simulink model "ndtm_V2"  (R2018b)
settings: configuration reference "Physics" (kept outside this file)
model workspace (MAT data in the model file):
  x0_initialstates = [0 0 0 0 0 0]
undefined symbols (not defined in the file): F0z, h, INIT__initialvalues__Vehicle_InitialPitchRate_radps, INIT__initialvalues__Vehicle_InitialRollRate_radps, INIT__initialvalues__Vehicle_InitialVelocity_mps__1, INIT__initialvalues__Vehicle_InitialVelocity_mps__2, INIT__initialvalues__Vehicle_InitialVelocity_mps__3, INIT__initialvalues__Vehicle_InitialYawRate_radps, SUS__Antisway__c_AntiSwayTSpringFrRe_Nmprad__1, SUS__Antisway__c_AntiSwayTSpringFrRe_Nmprad__2, SUS__Antisway__phi_AntiSwayNeutralAngleFrRe_rad__1, SUS__Antisway__phi_AntiSwayNeutralAngleFrRe_rad__2, SUS__Antisway__r_AntiSwayArmRadiusFrRe_m__1, SUS__Antisway__r_AntiSwayArmRadiusFrRe_m__2, SUS__Compliance__Cz_DamperRateFrRe_Nspm__1, SUS__Compliance__Cz_DamperRateFrRe_Nspm__2, SUS__Compliance__cz_SpringRateFrRe_Npm__1, SUS__Compliance__cz_SpringRateFrRe_Npm__2, SUS__Compliance__F0z_SpringPreloadFrRe_N__1, SUS__Compliance__F0z_SpringPreloadFrRe_N__2, SUS__Compliance__h_InertialFrameOffset_COGtoAxle_m, SUS__Kinematics__k_CamberATSteerCenterF__1, SUS__Kinematics__k_CamberATSteerCenterF__2, SUS__Kinematics__k_CamberVSHeightFrRe__1, SUS__Kinematics__k_CamberVSHeightFrRe__2, SUS__Kinematics__k_CasterATSteerCenterF__1, SUS__Kinematics__k_CasterATSteerCenterF__2, SUS__Kinematics__k_CasterVSHeightFrRe__1, SUS__Kinematics__k_CasterVSHeightFrRe__2, SUS__Kinematics__k_RollSteerVSHeightFrRe_radpm__1, SUS__Kinematics__k_RollSteerVSHeightFrRe_radpm__2, SUS__Kinematics__nu0_ToeATSteerCenterFrRe_rad__1, SUS__Kinematics__nu0_ToeATSteerCenterFrRe_rad__2, tireFL__SCALING__LFZO, tireFR__SCALING__LFZO, tireRL__SCALING__LFZO, tireRR__SCALING__LFZO, VEH, VEH__Aerodynamics__beta_wind_end_rad, VEH__Aerodynamics__beta_wind_start_rad, VEH__Aerodynamics__beta_wind_step_rad, VEH__Aerodynamics__cl_LongitudinalLift, VEH__Aerodynamics__Cs_LatDragCoeff_end, VEH__Aerodynamics__Cs_LatDragCoeff_start, VEH__Aerodynamics__Cs_LatDragCoeff_step, VEH__Aerodynamics__Cym_DragYawMomentCoeff_end, VEH__Aerodynamics__Cym_DragYawMomentCoeff_start, VEH__Aerodynamics__Cym_DragYawMomentCoeff_step, VEH__Environment__a_Gravity_mps2, VEH__Tires__p_Tires_pa__1, VEH__Tires__p_Tires_pa__2, VEH__Tires__p_Tires_pa__3, VEH__Tires__p_Tires_pa__4, VEH__VehicleData__l_WheelbaseF_m, VEH__VehicleData__l_WheelbaseTotal_m, VEH__VehicleData__m_Vehicle_kg, VEH__VehicleData__w_GeomCenterlineToCOG_m, VEH__VehicleData__w_TrackF_m, VEH__VehicleData__w_TrackR_m
libraries: vehdynlibsuspension x7, vehdynlibtire x4, vehdynlibtire_TUM x4, autolibutils x2, sharedtransform x2, vehdynlibeom_TUM x1
(part 3 of 4)

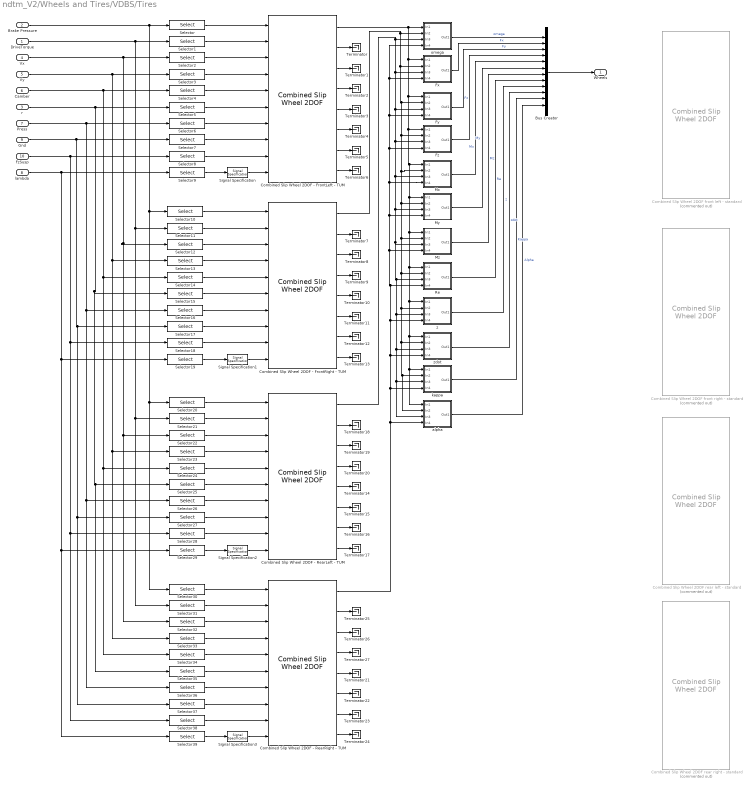
== system ndtm_V2/Wheels and Tires/VDBS/Tires ==
  DriveTorque : Inport
  Brake Pressure : Inport  Port=2
  r : Inport  Port=3
  Vx : Inport  Port=4
  Vy : Inport  Port=5
  Camber : Inport  Port=6
  Press : Inport  Port=7  Unit=Pa
  lambda : Inport  Port=8  Unit=1
  Gnd : Inport  Port=9
  FzSusp : Inport  Port=10
  Bus Creator : BusCreator  Inputs=12
  Combined Slip Wheel 2DOF front left - standard : vehdynlibtire/Combined Slip Wheel 2DOF  Commented=on  BrakeType=Disc  mu_static=0.6  mu_kinetic=0.6  disk_abore=.08  Rm=0.1475  num_pads=1  drum_abore=0.0508  drum_a=0.123  drum_c=0.212  drum_r=0.15  drum_theta1=0  drum_theta2=126  brake_p_bpt=[1 11.4736842105263 21.9473684210526 32.4210526315789 42.8947368421053 53.3684210526316 63.8421052631579 74.3157894736842 84.7894736842105 95.2631578947368 105.736842105263 116.210526315789 126.684210526316 137.157894736842 147.631578947368 158.105263157895 168.578947368421 179.052631578947 189.526315789474 200]  brake_n_bpt=[0 52.6315789473684 105.263157894737 157.894736842105 210.526315789474 263.157894736842 315.789473684211 368.421052631579 421.052631578947 473.684210526316 526.315789473684 578.947368421053 631.578947368421 684.210526315789 736.842105263158 789.473684210526 842.105263157895 894.736842105263 947.368421052632 1000]  f_brake_t=[43.4900602404453 42.5056030554862 41.5350898940194 40.5780454442085 39.6340111501808 38.7025443887544 37.7832176914519 36.8756180088306 35.9793460143796 35.0940154454303 34.2192524787115 33.3546951383474 32.4999927342521 31.6548053290159 30.8188032315107 29.991666515561 29.1730845621415 28.362755623661 27.5603864089927 26.765691687993;498.991217495636 487.695866636631 476.560505099801 465.579679307235 454.748127933653 444.060772460445 433.51270824929 423.099196101319 412.81565427025 402.657650900201 392.620896861006 382.701238955775 372.894653477208 363.197240090814 353.605216024701 344.114910546964 334.722759712992 325.425301366216 316.219170376863 307.10109410434;954.492374750826 932.886130217776 911.585920305583 890.581313170261 869.862244717126 849.419000532136 829.242198807128 809.322774193808 789.651962526121 770.221286354971 751.0225412433 732.047782773203 713.289314220164 694.739674852612 676.391628817892 658.238154578366 640.272434863842 622.48784710877 604.877954344734 587.436496520688;1409.99353200602 1378.07639379892 1346.61133551136 1315.58294703329 1284.9763615006 1254.77722860383 1224.97168936497 1195.5463522863 1166.48827078199 1137.78492180974 1109.42418562559 1081.39432659063 1053.68397496312 1026.28210961441 999.178041611083 972.361398609768 945.822110014692 919.550392851325 893.536738312604 867.771898937035;1865.49468926121 1823.26665738007 1781.63675071715 1740.58458089631 1700.09047828407 1660.13545667552 1620.7011799228 1581.76993037878 1543.32457903786 1505.34855726451 1467.82583000789 1430.74087040806 1394.07863570608 1357.82454437621 1321.96445440427 1286.48464264117 1251.37178516554 1216.61293859388 1182.19552228048 1148.10730135338;2320.9958465164 2268.45692096121 2216.66216592293 2165.58621475934 2115.20459506754 2065.49368474721 2016.43067048064 1967.99350847127 1920.16088729373 1872.91219271928 1826.22747439018 1780.08741422549 1734.47329644903 1689.36697913801 1644.75086719747 1600.60788667257 1556.92146031639 1513.67548433643 1470.85430624835 1428.44270376973;2776.49700377159 2713.64718454235 2651.68758112871 2590.58784862237 2530.31871185102 2470.8519128189 2412.16016103848 2354.21708656376 2296.9971955496 2240.47582817405 2184.62911877248 2129.43395804292 2074.86795719199 2020.9094138998 1967.53727999066 1914.73113070398 1862.47113546724 1810.73803007899 1759.51309021622 1708.77810618608;3231.99816102678 3158.8374481235 3086.71299633449 3015.58948248539 2945.43282863449 2876.21014089059 2807.88965159632 2740.44066465625 2673.83350380547 2608.03946362882 2543.03076315477 2478.78050186034 2415.26261793494 2352.4518486616 2290.32369278385 2228.85437473538 2168.02081061809 2107.80057582154 2048.17187418409 1989.11350860242;3687.49931828197 3604.02771170464 3521.73841154027 3440.59111634842 3360.54694541796 3281.56836896228 3203.61914215416 3126.66424274874 3050.66981206134 2975.60309908359 2901.43240753707 2828.12704567777 2755.6572786779 2683.9942834234 2613.11010557704 2542.97761876678 2473.57048576894 2404.8631215641 2336.83065815196 2269.44891101877;4143.00047553716 4049.21797528579 3956.76382674606 3865.59275021144 3775.66106220143 3686.92659703397 3599.34863271199 3512.88782084123 3427.50612031721 3343.16673453836 3259.83405191936 3177.4735894952 3096.05193942085 3015.5367181852 2935.89651837023 2857.10086279818 2779.12016091979 2701.92566730665 2625.48944211983 2549.78431343512;4598.50163279235 4494.40823886693 4391.78924195184 4290.59438407447 4190.77517898491 4092.28482510566 3995.07812326983 3899.11139893372 3804.34242857308 3710.73036999313 3618.23569630166 3526.82013331263 3436.44660016381 3347.079152947 3258.68293116342 3171.22410682959 3084.66983607064 2998.98821304921 2914.1482260877 2830.11971585147;5054.00279004754 4939.59850244808 4826.81465715762 4715.59601793749 4605.88929576838 4497.64305317735 4390.80761382767 4285.3349770262 4181.17873682896 4078.2940054479 3976.63734068395 3876.16667713006 3776.84126090677 3678.62158770879 3581.46934395661 3485.34735086099 ...(+2764 chars)]  tireParamSet=vdynPassCar.mat  plySteer=off  turnslip=off  PRESMAX=1000000  PRESMIN=10000  FZMAX=10000  FZMIN=100  VXLOW=0.1  KPUMAX=1.5  KPUMIN=-1.5  ALPMAX=1.5  ALPMIN=-1.5  CAMMAX=0.2  CAMMIN=-0.2  LONGVL=16.7  omegao=0  br=1e-3  UNLOADED_RADIUS=0.42  NOMPRES=224000  FNOMIN=4000  WIDTH=0.209  MASS=9.46+20  IYY=0.740633832792491  GRAVITY=-9.81  zo=.015  zdoto=0  BREFF=8.25094594147963  DREFF=0.260468730454265  FREFF=0.0735298544471851  Q_RE0=1.00866439868088  Q_V1=0.000760413786224011  Q_V2=0.0463384792019201  Q_FZ1=0  Q_FZ2=15.6870832810226  Q_FZ3=0  Q_FCX=0.138643970247602  Q_FCY=0.10843499565426  Q_FCY2=-0.465763352339538  PFZ1=0.69958166705601  VERTICAL_STIFFNESS=207885.061134007  VERTICAL_DAMPING=494.649255786991  LONGITUDINAL_STIFFNESS=388714.175879854  LATERAL_STIFFNESS=157087.404633332  PCFX1=0.18539229191199  PCFX2=0  PCFX3=0  PCFY1=0.163183345037677  PCFY2=0  PCFY3=0.249094918231954  Q_RA1=0.675942571700787  Q_RA2=0.73800463546164  Q_RB1=1.04487486456705  Q_RB2=-1.191763806629  PCX1=1.58523057950359  PDX1=1.0239116238178  PDX2=-0.0842405110022724  PDX3=0  PEX1=0.110312777158455  PEX2=0.313468516038146  PEX3=0  PEX4=0.0016060905760045  PKX1=21.3872544684023  PKX2=14.0006541873175  PKX3=-0.405326109653452  PHX1=0.000212599305364818  PHX2=0.00115950515263055  PVX1=1.59236164471432e-05  PVX2=0.000104321112127671  PPX1=-0.349461321276586  PPX2=0.387840040616429  PPX3=-0.0969947336569324  PPX4=0.0632271859795801  RBX1=12.7633329850276  RBX2=9.5787123658471  RBX3=0  RCX1=1.02796280922059  REX1=-0.45202516851367  REX2=-0.47304886171176  RHX1=0.000233272373115809  QSX1=-0.00788307788961443  QSX2=0.954629515459396  QSX3=0.0155855777667025  QSX4=0.125904607142414  QSX5=1.01110069703963  QSX6=20.1938577118433  QSX7=0.310818120717083  QSX8=-0.0430823751139655  QSX9=0.636494404888216  QSX10=0.142438060591663  QSX11=0.346766530036373  QSX12=0  QSX13=0  QSX14=0  PPMX1=0  PCY1=1.34299950037631  PDY1=0.878267729082195  PDY2=-0.0644597923147385  PDY3=0  PEY1=-0.809776534470972  PEY2=-0.600180598867198  PEY3=0.0991732552633487  PEY4=-6.5577974035573  PEY5=0  PKY1=-15.57  PKY2=1.73126522291751  PKY3=0.365349873517229  PKY4=1.98176755955416  PKY5=0  PKY6=-0.884005199550313  PKY7=-0.237259727611847  PHY1=-0.00183370557235628  PHY2=0.00346401302716671  PVY1=-0.00675427560163264  PVY2=0.036379218103843  PVY3=-0.163543984089166  PVY4=-0.491003349625726  PPY1=-0.62059646553185  PPY2=-0.0647824842338686  PPY3=-0.164648843290686  PPY4=0.283193909060098  PPY5=0  RBY1=10.7588809173639  RBY2=7.70420065295029  RBY3=3.40283755070691e-06  RBY4=0  RCY1=1.06691874059059  REY1=0.308244924574305  REY2=7.48775032604508e-06  RHY1=0.0118479204960415  RHY2=7.63650177161071e-06  RVY1=0.0560024425050078  RVY2=7.48487127056197e-06  RVY3=0  RVY4=98.4047026517149  RVY5=2.02759273900054  RVY6=15.7623064923347  QSY1=0.00699077564863536  QSY2=0  QSY3=0.00153535478298811  QSY4=8.55710322455322e-05  QSY5=0  QSY6=0  QSY7=0.89443879773793  QSY8=-0.403227641260894  QBZ1=11.666656027484  QBZ2=-1.30355438574485  QBZ3=0  QBZ4=0.177918305399071  QBZ5=-0.162481135068033  QBZ6=0  QBZ9=30.1445534682089  QBZ10=0  QCZ1=1.29026978207574  QDZ1=0.0886972644991399  QDZ2=-0.0058634820161856  QDZ3=0.3805597481383  QDZ4=0  QDZ6=0.00160914918118959  QDZ7=-0.00211036330862154  QDZ8=-0.13921904912557  QDZ9=0.00816585550028243  QDZ10=0  QDZ11=0  QEZ1=-2.19802254534746  QEZ2=1.01850535789165  QEZ3=0  QEZ4=0.278379679112054  QEZ5=-0.548414722765386  QHZ1=0.00148361198869669  QHZ2=0.00202017567585904  QHZ3=0.240316641332066  QHZ4=-0.210114035738085  PPZ1=-0.443927982388615  PPZ2=0  SSZ1=0.00914999585397887  SSZ2=0.0389830656052735  SSZ3=0  SSZ4=0  PDXP1=0.396718274678791  PDXP2=0  PDXP3=0  PKYP1=1.00587060633573  PDYP1=0.40483048923438  PDYP2=0  PDYP3=0  PDYP4=0  PHYP1=0.992731942067188  PHYP2=0.150352945499914  PHYP3=0  PHYP4=-3.98988682633674  PECP1=0.502379254513503  PECP2=0  QDTP1=10.0178654287947  QCRP1=0.200627747200702  QCRP2=0.0995735881599772  QBRP1=0.0997107127960717  QDRP1=1.01432910167423  QDRP2=0  aMode=2
      settings: SourceProductName=Vehicle Dynamics Blockset
  Combined Slip Wheel 2DOF front right - standard : vehdynlibtire/Combined Slip Wheel 2DOF  Commented=on  BrakeType=Disc  mu_static=0.6  mu_kinetic=0.6  disk_abore=0.08  Rm=0.1475  num_pads=1  drum_abore=0.0508  drum_a=0.123  drum_c=0.212  drum_r=0.15  drum_theta1=0  drum_theta2=126  brake_p_bpt=[1 11.4736842105263 21.9473684210526 32.4210526315789 42.8947368421053 53.3684210526316 63.8421052631579 74.3157894736842 84.7894736842105 95.2631578947368 105.736842105263 116.210526315789 126.684210526316 137.157894736842 147.631578947368 158.105263157895 168.578947368421 179.052631578947 189.526315789474 200]  brake_n_bpt=[0 52.6315789473684 105.263157894737 157.894736842105 210.526315789474 263.157894736842 315.789473684211 368.421052631579 421.052631578947 473.684210526316 526.315789473684 578.947368421053 631.578947368421 684.210526315789 736.842105263158 789.473684210526 842.105263157895 894.736842105263 947.368421052632 1000]  f_brake_t=[43.4900602404453 42.5056030554862 41.5350898940194 40.5780454442085 39.6340111501808 38.7025443887544 37.7832176914519 36.8756180088306 35.9793460143796 35.0940154454303 34.2192524787115 33.3546951383474 32.4999927342521 31.6548053290159 30.8188032315107 29.991666515561 29.1730845621415 28.362755623661 27.5603864089927 26.765691687993;498.991217495636 487.695866636631 476.560505099801 465.579679307235 454.748127933653 444.060772460445 433.51270824929 423.099196101319 412.81565427025 402.657650900201 392.620896861006 382.701238955775 372.894653477208 363.197240090814 353.605216024701 344.114910546964 334.722759712992 325.425301366216 316.219170376863 307.10109410434;954.492374750826 932.886130217776 911.585920305583 890.581313170261 869.862244717126 849.419000532136 829.242198807128 809.322774193808 789.651962526121 770.221286354971 751.0225412433 732.047782773203 713.289314220164 694.739674852612 676.391628817892 658.238154578366 640.272434863842 622.48784710877 604.877954344734 587.436496520688;1409.99353200602 1378.07639379892 1346.61133551136 1315.58294703329 1284.9763615006 1254.77722860383 1224.97168936497 1195.5463522863 1166.48827078199 1137.78492180974 1109.42418562559 1081.39432659063 1053.68397496312 1026.28210961441 999.178041611083 972.361398609768 945.822110014692 919.550392851325 893.536738312604 867.771898937035;1865.49468926121 1823.26665738007 1781.63675071715 1740.58458089631 1700.09047828407 1660.13545667552 1620.7011799228 1581.76993037878 1543.32457903786 1505.34855726451 1467.82583000789 1430.74087040806 1394.07863570608 1357.82454437621 1321.96445440427 1286.48464264117 1251.37178516554 1216.61293859388 1182.19552228048 1148.10730135338;2320.9958465164 2268.45692096121 2216.66216592293 2165.58621475934 2115.20459506754 2065.49368474721 2016.43067048064 1967.99350847127 1920.16088729373 1872.91219271928 1826.22747439018 1780.08741422549 1734.47329644903 1689.36697913801 1644.75086719747 1600.60788667257 1556.92146031639 1513.67548433643 1470.85430624835 1428.44270376973;2776.49700377159 2713.64718454235 2651.68758112871 2590.58784862237 2530.31871185102 2470.8519128189 2412.16016103848 2354.21708656376 2296.9971955496 2240.47582817405 2184.62911877248 2129.43395804292 2074.86795719199 2020.9094138998 1967.53727999066 1914.73113070398 1862.47113546724 1810.73803007899 1759.51309021622 1708.77810618608;3231.99816102678 3158.8374481235 3086.71299633449 3015.58948248539 2945.43282863449 2876.21014089059 2807.88965159632 2740.44066465625 2673.83350380547 2608.03946362882 2543.03076315477 2478.78050186034 2415.26261793494 2352.4518486616 2290.32369278385 2228.85437473538 2168.02081061809 2107.80057582154 2048.17187418409 1989.11350860242;3687.49931828197 3604.02771170464 3521.73841154027 3440.59111634842 3360.54694541796 3281.56836896228 3203.61914215416 3126.66424274874 3050.66981206134 2975.60309908359 2901.43240753707 2828.12704567777 2755.6572786779 2683.9942834234 2613.11010557704 2542.97761876678 2473.57048576894 2404.8631215641 2336.83065815196 2269.44891101877;4143.00047553716 4049.21797528579 3956.76382674606 3865.59275021144 3775.66106220143 3686.92659703397 3599.34863271199 3512.88782084123 3427.50612031721 3343.16673453836 3259.83405191936 3177.4735894952 3096.05193942085 3015.5367181852 2935.89651837023 2857.10086279818 2779.12016091979 2701.92566730665 2625.48944211983 2549.78431343512;4598.50163279235 4494.40823886693 4391.78924195184 4290.59438407447 4190.77517898491 4092.28482510566 3995.07812326983 3899.11139893372 3804.34242857308 3710.73036999313 3618.23569630166 3526.82013331263 3436.44660016381 3347.079152947 3258.68293116342 3171.22410682959 3084.66983607064 2998.98821304921 2914.1482260877 2830.11971585147;5054.00279004754 4939.59850244808 4826.81465715762 4715.59601793749 4605.88929576838 4497.64305317735 4390.80761382767 4285.3349770262 4181.17873682896 4078.2940054479 3976.63734068395 3876.16667713006 3776.84126090677 3678.62158770879 3581.46934395661 3485.34735086099 ...(+2764 chars)]  tireParamSet=vdynPassCar.mat  plySteer=off  turnslip=off  PRESMAX=1000000  PRESMIN=10000  FZMAX=10000  FZMIN=100  VXLOW=0.1  KPUMAX=1.5  KPUMIN=-1.5  ALPMAX=1.5  ALPMIN=-1.5  CAMMAX=0.2  CAMMIN=-0.2  LONGVL=16.7  omegao=0  br=1e-3  UNLOADED_RADIUS=0.42  NOMPRES=224000  FNOMIN=4000  WIDTH=0.209  MASS=9.46+20  IYY=0.740633832792491  GRAVITY=-9.81  zo=.015  zdoto=0  BREFF=8.25094594147963  DREFF=0.260468730454265  FREFF=0.0735298544471851  Q_RE0=1.00866439868088  Q_V1=0.000760413786224011  Q_V2=0.0463384792019201  Q_FZ1=0  Q_FZ2=15.6870832810226  Q_FZ3=0  Q_FCX=0.138643970247602  Q_FCY=0.10843499565426  Q_FCY2=-0.465763352339538  PFZ1=0.69958166705601  VERTICAL_STIFFNESS=207885.061134007  VERTICAL_DAMPING=494.649255786991  LONGITUDINAL_STIFFNESS=388714.175879854  LATERAL_STIFFNESS=157087.404633332  PCFX1=0.18539229191199  PCFX2=0  PCFX3=0  PCFY1=0.163183345037677  PCFY2=0  PCFY3=0.249094918231954  Q_RA1=0.675942571700787  Q_RA2=0.73800463546164  Q_RB1=1.04487486456705  Q_RB2=-1.191763806629  PCX1=1.58523057950359  PDX1=1.0239116238178  PDX2=-0.0842405110022724  PDX3=0  PEX1=0.110312777158455  PEX2=0.313468516038146  PEX3=0  PEX4=0.0016060905760045  PKX1=21.3872544684023  PKX2=14.0006541873175  PKX3=-0.405326109653452  PHX1=0.000212599305364818  PHX2=0.00115950515263055  PVX1=1.59236164471432e-05  PVX2=0.000104321112127671  PPX1=-0.349461321276586  PPX2=0.387840040616429  PPX3=-0.0969947336569324  PPX4=0.0632271859795801  RBX1=12.7633329850276  RBX2=9.5787123658471  RBX3=0  RCX1=1.02796280922059  REX1=-0.45202516851367  REX2=-0.47304886171176  RHX1=0.000233272373115809  QSX1=-0.00788307788961443  QSX2=0.954629515459396  QSX3=0.0155855777667025  QSX4=0.125904607142414  QSX5=1.01110069703963  QSX6=20.1938577118433  QSX7=0.310818120717083  QSX8=-0.0430823751139655  QSX9=0.636494404888216  QSX10=0.142438060591663  QSX11=0.346766530036373  QSX12=0  QSX13=0  QSX14=0  PPMX1=0  PCY1=1.34299950037631  PDY1=0.878267729082195  PDY2=-0.0644597923147385  PDY3=0  PEY1=-0.809776534470972  PEY2=-0.600180598867198  PEY3=0.0991732552633487  PEY4=-6.5577974035573  PEY5=0  PKY1=-15.57  PKY2=1.73126522291751  PKY3=0.365349873517229  PKY4=1.98176755955416  PKY5=0  PKY6=-0.884005199550313  PKY7=-0.237259727611847  PHY1=-0.00183370557235628  PHY2=0.00346401302716671  PVY1=-0.00675427560163264  PVY2=0.036379218103843  PVY3=-0.163543984089166  PVY4=-0.491003349625726  PPY1=-0.62059646553185  PPY2=-0.0647824842338686  PPY3=-0.164648843290686  PPY4=0.283193909060098  PPY5=0  RBY1=10.7588809173639  RBY2=7.70420065295029  RBY3=3.40283755070691e-06  RBY4=0  RCY1=1.06691874059059  REY1=0.308244924574305  REY2=7.48775032604508e-06  RHY1=0.0118479204960415  RHY2=7.63650177161071e-06  RVY1=0.0560024425050078  RVY2=7.48487127056197e-06  RVY3=0  RVY4=98.4047026517149  RVY5=2.02759273900054  RVY6=15.7623064923347  QSY1=0.00699077564863536  QSY2=0  QSY3=0.00153535478298811  QSY4=8.55710322455322e-05  QSY5=0  QSY6=0  QSY7=0.89443879773793  QSY8=-0.403227641260894  QBZ1=11.666656027484  QBZ2=-1.30355438574485  QBZ3=0  QBZ4=0.177918305399071  QBZ5=-0.162481135068033  QBZ6=0  QBZ9=30.1445534682089  QBZ10=0  QCZ1=1.29026978207574  QDZ1=0.0886972644991399  QDZ2=-0.0058634820161856  QDZ3=0.3805597481383  QDZ4=0  QDZ6=0.00160914918118959  QDZ7=-0.00211036330862154  QDZ8=-0.13921904912557  QDZ9=0.00816585550028243  QDZ10=0  QDZ11=0  QEZ1=-2.19802254534746  QEZ2=1.01850535789165  QEZ3=0  QEZ4=0.278379679112054  QEZ5=-0.548414722765386  QHZ1=0.00148361198869669  QHZ2=0.00202017567585904  QHZ3=0.240316641332066  QHZ4=-0.210114035738085  PPZ1=-0.443927982388615  PPZ2=0  SSZ1=0.00914999585397887  SSZ2=0.0389830656052735  SSZ3=0  SSZ4=0  PDXP1=0.396718274678791  PDXP2=0  PDXP3=0  PKYP1=1.00587060633573  PDYP1=0.40483048923438  PDYP2=0  PDYP3=0  PDYP4=0  PHYP1=0.992731942067188  PHYP2=0.150352945499914  PHYP3=0  PHYP4=-3.98988682633674  PECP1=0.502379254513503  PECP2=0  QDTP1=10.0178654287947  QCRP1=0.200627747200702  QCRP2=0.0995735881599772  QBRP1=0.0997107127960717  QDRP1=1.01432910167423  QDRP2=0  aMode=2
      settings: SourceProductName=Vehicle Dynamics Blockset
  Combined Slip Wheel 2DOF rear left - standard : vehdynlibtire/Combined Slip Wheel 2DOF  Commented=on  BrakeType=Disc  mu_static=0.6  mu_kinetic=0.6  disk_abore=0.08  Rm=0.1475  num_pads=1  drum_abore=0.0508  drum_a=0.123  drum_c=0.212  drum_r=0.15  drum_theta1=0  drum_theta2=126  brake_p_bpt=[1 11.4736842105263 21.9473684210526 32.4210526315789 42.8947368421053 53.3684210526316 63.8421052631579 74.3157894736842 84.7894736842105 95.2631578947368 105.736842105263 116.210526315789 126.684210526316 137.157894736842 147.631578947368 158.105263157895 168.578947368421 179.052631578947 189.526315789474 200]  brake_n_bpt=[0 52.6315789473684 105.263157894737 157.894736842105 210.526315789474 263.157894736842 315.789473684211 368.421052631579 421.052631578947 473.684210526316 526.315789473684 578.947368421053 631.578947368421 684.210526315789 736.842105263158 789.473684210526 842.105263157895 894.736842105263 947.368421052632 1000]  f_brake_t=[43.4900602404453 42.5056030554862 41.5350898940194 40.5780454442085 39.6340111501808 38.7025443887544 37.7832176914519 36.8756180088306 35.9793460143796 35.0940154454303 34.2192524787115 33.3546951383474 32.4999927342521 31.6548053290159 30.8188032315107 29.991666515561 29.1730845621415 28.362755623661 27.5603864089927 26.765691687993;498.991217495636 487.695866636631 476.560505099801 465.579679307235 454.748127933653 444.060772460445 433.51270824929 423.099196101319 412.81565427025 402.657650900201 392.620896861006 382.701238955775 372.894653477208 363.197240090814 353.605216024701 344.114910546964 334.722759712992 325.425301366216 316.219170376863 307.10109410434;954.492374750826 932.886130217776 911.585920305583 890.581313170261 869.862244717126 849.419000532136 829.242198807128 809.322774193808 789.651962526121 770.221286354971 751.0225412433 732.047782773203 713.289314220164 694.739674852612 676.391628817892 658.238154578366 640.272434863842 622.48784710877 604.877954344734 587.436496520688;1409.99353200602 1378.07639379892 1346.61133551136 1315.58294703329 1284.9763615006 1254.77722860383 1224.97168936497 1195.5463522863 1166.48827078199 1137.78492180974 1109.42418562559 1081.39432659063 1053.68397496312 1026.28210961441 999.178041611083 972.361398609768 945.822110014692 919.550392851325 893.536738312604 867.771898937035;1865.49468926121 1823.26665738007 1781.63675071715 1740.58458089631 1700.09047828407 1660.13545667552 1620.7011799228 1581.76993037878 1543.32457903786 1505.34855726451 1467.82583000789 1430.74087040806 1394.07863570608 1357.82454437621 1321.96445440427 1286.48464264117 1251.37178516554 1216.61293859388 1182.19552228048 1148.10730135338;2320.9958465164 2268.45692096121 2216.66216592293 2165.58621475934 2115.20459506754 2065.49368474721 2016.43067048064 1967.99350847127 1920.16088729373 1872.91219271928 1826.22747439018 1780.08741422549 1734.47329644903 1689.36697913801 1644.75086719747 1600.60788667257 1556.92146031639 1513.67548433643 1470.85430624835 1428.44270376973;2776.49700377159 2713.64718454235 2651.68758112871 2590.58784862237 2530.31871185102 2470.8519128189 2412.16016103848 2354.21708656376 2296.9971955496 2240.47582817405 2184.62911877248 2129.43395804292 2074.86795719199 2020.9094138998 1967.53727999066 1914.73113070398 1862.47113546724 1810.73803007899 1759.51309021622 1708.77810618608;3231.99816102678 3158.8374481235 3086.71299633449 3015.58948248539 2945.43282863449 2876.21014089059 2807.88965159632 2740.44066465625 2673.83350380547 2608.03946362882 2543.03076315477 2478.78050186034 2415.26261793494 2352.4518486616 2290.32369278385 2228.85437473538 2168.02081061809 2107.80057582154 2048.17187418409 1989.11350860242;3687.49931828197 3604.02771170464 3521.73841154027 3440.59111634842 3360.54694541796 3281.56836896228 3203.61914215416 3126.66424274874 3050.66981206134 2975.60309908359 2901.43240753707 2828.12704567777 2755.6572786779 2683.9942834234 2613.11010557704 2542.97761876678 2473.57048576894 2404.8631215641 2336.83065815196 2269.44891101877;4143.00047553716 4049.21797528579 3956.76382674606 3865.59275021144 3775.66106220143 3686.92659703397 3599.34863271199 3512.88782084123 3427.50612031721 3343.16673453836 3259.83405191936 3177.4735894952 3096.05193942085 3015.5367181852 2935.89651837023 2857.10086279818 2779.12016091979 2701.92566730665 2625.48944211983 2549.78431343512;4598.50163279235 4494.40823886693 4391.78924195184 4290.59438407447 4190.77517898491 4092.28482510566 3995.07812326983 3899.11139893372 3804.34242857308 3710.73036999313 3618.23569630166 3526.82013331263 3436.44660016381 3347.079152947 3258.68293116342 3171.22410682959 3084.66983607064 2998.98821304921 2914.1482260877 2830.11971585147;5054.00279004754 4939.59850244808 4826.81465715762 4715.59601793749 4605.88929576838 4497.64305317735 4390.80761382767 4285.3349770262 4181.17873682896 4078.2940054479 3976.63734068395 3876.16667713006 3776.84126090677 3678.62158770879 3581.46934395661 3485.34735086099 ...(+2764 chars)]  tireParamSet=vdynPassCar.mat  plySteer=off  turnslip=off  PRESMAX=1000000  PRESMIN=10000  FZMAX=10000  FZMIN=100  VXLOW=0.1  KPUMAX=1.5  KPUMIN=-1.5  ALPMAX=1.5  ALPMIN=-1.5  CAMMAX=0.2  CAMMIN=-0.2  LONGVL=16.7  omegao=0  br=1e-3  UNLOADED_RADIUS=0.42  NOMPRES=224000  FNOMIN=4000  WIDTH=0.209  MASS=9.46+20  IYY=0.740633832792491  GRAVITY=-9.81  zo=.015  zdoto=0  BREFF=8.25094594147963  DREFF=0.260468730454265  FREFF=0.0735298544471851  Q_RE0=1.00866439868088  Q_V1=0.000760413786224011  Q_V2=0.0463384792019201  Q_FZ1=0  Q_FZ2=15.6870832810226  Q_FZ3=0  Q_FCX=0.138643970247602  Q_FCY=0.10843499565426  Q_FCY2=-0.465763352339538  PFZ1=0.69958166705601  VERTICAL_STIFFNESS=207885.061134007  VERTICAL_DAMPING=494.649255786991  LONGITUDINAL_STIFFNESS=388714.175879854  LATERAL_STIFFNESS=157087.404633332  PCFX1=0.18539229191199  PCFX2=0  PCFX3=0  PCFY1=0.163183345037677  PCFY2=0  PCFY3=0.249094918231954  Q_RA1=0.675942571700787  Q_RA2=0.73800463546164  Q_RB1=1.04487486456705  Q_RB2=-1.191763806629  PCX1=1.58523057950359  PDX1=1.0239116238178  PDX2=-0.0842405110022724  PDX3=0  PEX1=0.110312777158455  PEX2=0.313468516038146  PEX3=0  PEX4=0.0016060905760045  PKX1=21.3872544684023  PKX2=14.0006541873175  PKX3=-0.405326109653452  PHX1=0.000212599305364818  PHX2=0.00115950515263055  PVX1=1.59236164471432e-05  PVX2=0.000104321112127671  PPX1=-0.349461321276586  PPX2=0.387840040616429  PPX3=-0.0969947336569324  PPX4=0.0632271859795801  RBX1=12.7633329850276  RBX2=9.5787123658471  RBX3=0  RCX1=1.02796280922059  REX1=-0.45202516851367  REX2=-0.47304886171176  RHX1=0.000233272373115809  QSX1=-0.00788307788961443  QSX2=0.954629515459396  QSX3=0.0155855777667025  QSX4=0.125904607142414  QSX5=1.01110069703963  QSX6=20.1938577118433  QSX7=0.310818120717083  QSX8=-0.0430823751139655  QSX9=0.636494404888216  QSX10=0.142438060591663  QSX11=0.346766530036373  QSX12=0  QSX13=0  QSX14=0  PPMX1=0  PCY1=1.34299950037631  PDY1=0.878267729082195  PDY2=-0.0644597923147385  PDY3=0  PEY1=-0.809776534470972  PEY2=-0.600180598867198  PEY3=0.0991732552633487  PEY4=-6.5577974035573  PEY5=0  PKY1=-15.5714726518315  PKY2=1.73126522291751  PKY3=0.365349873517229  PKY4=1.98176755955416  PKY5=0  PKY6=-0.884005199550313  PKY7=-0.237259727611847  PHY1=-0.00183370557235628  PHY2=0.00346401302716671  PVY1=-0.00675427560163264  PVY2=0.036379218103843  PVY3=-0.163543984089166  PVY4=-0.491003349625726  PPY1=-0.62059646553185  PPY2=-0.0647824842338686  PPY3=-0.164648843290686  PPY4=0.283193909060098  PPY5=0  RBY1=10.7588809173639  RBY2=7.70420065295029  RBY3=3.40283755070691e-06  RBY4=0  RCY1=1.06691874059059  REY1=0.308244924574305  REY2=7.48775032604508e-06  RHY1=0.0118479204960415  RHY2=7.63650177161071e-06  RVY1=0.0560024425050078  RVY2=7.48487127056197e-06  RVY3=0  RVY4=98.4047026517149  RVY5=2.02759273900054  RVY6=15.7623064923347  QSY1=0.00699077564863536  QSY2=0  QSY3=0.00153535478298811  QSY4=8.55710322455322e-05  QSY5=0  QSY6=0  QSY7=0.89443879773793  QSY8=-0.403227641260894  QBZ1=11.666656027484  QBZ2=-1.30355438574485  QBZ3=0  QBZ4=0.177918305399071  QBZ5=-0.162481135068033  QBZ6=0  QBZ9=30.1445534682089  QBZ10=0  QCZ1=1.29026978207574  QDZ1=0.0886972644991399  QDZ2=-0.0058634820161856  QDZ3=0.3805597481383  QDZ4=0  QDZ6=0.00160914918118959  QDZ7=-0.00211036330862154  QDZ8=-0.13921904912557  QDZ9=0.00816585550028243  QDZ10=0  QDZ11=0  QEZ1=-2.19802254534746  QEZ2=1.01850535789165  QEZ3=0  QEZ4=0.278379679112054  QEZ5=-0.548414722765386  QHZ1=0.00148361198869669  QHZ2=0.00202017567585904  QHZ3=0.240316641332066  QHZ4=-0.210114035738085  PPZ1=-0.443927982388615  PPZ2=0  SSZ1=0.00914999585397887  SSZ2=0.0389830656052735  SSZ3=0  SSZ4=0  PDXP1=0.396718274678791  PDXP2=0  PDXP3=0  PKYP1=1.00587060633573  PDYP1=0.40483048923438  PDYP2=0  PDYP3=0  PDYP4=0  PHYP1=0.992731942067188  PHYP2=0.150352945499914  PHYP3=0  PHYP4=-3.98988682633674  PECP1=0.502379254513503  PECP2=0  QDTP1=10.0178654287947  QCRP1=0.200627747200702  QCRP2=0.0995735881599772  QBRP1=0.0997107127960717  QDRP1=1.01432910167423  QDRP2=0  aMode=2
      settings: SourceProductName=Vehicle Dynamics Blockset
  Combined Slip Wheel 2DOF rear right - standard : vehdynlibtire/Combined Slip Wheel 2DOF  Commented=on  BrakeType=Disc  mu_static=0.6  mu_kinetic=0.6  disk_abore=0.08  Rm=0.1475  num_pads=1  drum_abore=0.0508  drum_a=0.123  drum_c=0.212  drum_r=0.15  drum_theta1=0  drum_theta2=126  brake_p_bpt=[1 11.4736842105263 21.9473684210526 32.4210526315789 42.8947368421053 53.3684210526316 63.8421052631579 74.3157894736842 84.7894736842105 95.2631578947368 105.736842105263 116.210526315789 126.684210526316 137.157894736842 147.631578947368 158.105263157895 168.578947368421 179.052631578947 189.526315789474 200]  brake_n_bpt=[0 52.6315789473684 105.263157894737 157.894736842105 210.526315789474 263.157894736842 315.789473684211 368.421052631579 421.052631578947 473.684210526316 526.315789473684 578.947368421053 631.578947368421 684.210526315789 736.842105263158 789.473684210526 842.105263157895 894.736842105263 947.368421052632 1000]  f_brake_t=[43.4900602404453 42.5056030554862 41.5350898940194 40.5780454442085 39.6340111501808 38.7025443887544 37.7832176914519 36.8756180088306 35.9793460143796 35.0940154454303 34.2192524787115 33.3546951383474 32.4999927342521 31.6548053290159 30.8188032315107 29.991666515561 29.1730845621415 28.362755623661 27.5603864089927 26.765691687993;498.991217495636 487.695866636631 476.560505099801 465.579679307235 454.748127933653 444.060772460445 433.51270824929 423.099196101319 412.81565427025 402.657650900201 392.620896861006 382.701238955775 372.894653477208 363.197240090814 353.605216024701 344.114910546964 334.722759712992 325.425301366216 316.219170376863 307.10109410434;954.492374750826 932.886130217776 911.585920305583 890.581313170261 869.862244717126 849.419000532136 829.242198807128 809.322774193808 789.651962526121 770.221286354971 751.0225412433 732.047782773203 713.289314220164 694.739674852612 676.391628817892 658.238154578366 640.272434863842 622.48784710877 604.877954344734 587.436496520688;1409.99353200602 1378.07639379892 1346.61133551136 1315.58294703329 1284.9763615006 1254.77722860383 1224.97168936497 1195.5463522863 1166.48827078199 1137.78492180974 1109.42418562559 1081.39432659063 1053.68397496312 1026.28210961441 999.178041611083 972.361398609768 945.822110014692 919.550392851325 893.536738312604 867.771898937035;1865.49468926121 1823.26665738007 1781.63675071715 1740.58458089631 1700.09047828407 1660.13545667552 1620.7011799228 1581.76993037878 1543.32457903786 1505.34855726451 1467.82583000789 1430.74087040806 1394.07863570608 1357.82454437621 1321.96445440427 1286.48464264117 1251.37178516554 1216.61293859388 1182.19552228048 1148.10730135338;2320.9958465164 2268.45692096121 2216.66216592293 2165.58621475934 2115.20459506754 2065.49368474721 2016.43067048064 1967.99350847127 1920.16088729373 1872.91219271928 1826.22747439018 1780.08741422549 1734.47329644903 1689.36697913801 1644.75086719747 1600.60788667257 1556.92146031639 1513.67548433643 1470.85430624835 1428.44270376973;2776.49700377159 2713.64718454235 2651.68758112871 2590.58784862237 2530.31871185102 2470.8519128189 2412.16016103848 2354.21708656376 2296.9971955496 2240.47582817405 2184.62911877248 2129.43395804292 2074.86795719199 2020.9094138998 1967.53727999066 1914.73113070398 1862.47113546724 1810.73803007899 1759.51309021622 1708.77810618608;3231.99816102678 3158.8374481235 3086.71299633449 3015.58948248539 2945.43282863449 2876.21014089059 2807.88965159632 2740.44066465625 2673.83350380547 2608.03946362882 2543.03076315477 2478.78050186034 2415.26261793494 2352.4518486616 2290.32369278385 2228.85437473538 2168.02081061809 2107.80057582154 2048.17187418409 1989.11350860242;3687.49931828197 3604.02771170464 3521.73841154027 3440.59111634842 3360.54694541796 3281.56836896228 3203.61914215416 3126.66424274874 3050.66981206134 2975.60309908359 2901.43240753707 2828.12704567777 2755.6572786779 2683.9942834234 2613.11010557704 2542.97761876678 2473.57048576894 2404.8631215641 2336.83065815196 2269.44891101877;4143.00047553716 4049.21797528579 3956.76382674606 3865.59275021144 3775.66106220143 3686.92659703397 3599.34863271199 3512.88782084123 3427.50612031721 3343.16673453836 3259.83405191936 3177.4735894952 3096.05193942085 3015.5367181852 2935.89651837023 2857.10086279818 2779.12016091979 2701.92566730665 2625.48944211983 2549.78431343512;4598.50163279235 4494.40823886693 4391.78924195184 4290.59438407447 4190.77517898491 4092.28482510566 3995.07812326983 3899.11139893372 3804.34242857308 3710.73036999313 3618.23569630166 3526.82013331263 3436.44660016381 3347.079152947 3258.68293116342 3171.22410682959 3084.66983607064 2998.98821304921 2914.1482260877 2830.11971585147;5054.00279004754 4939.59850244808 4826.81465715762 4715.59601793749 4605.88929576838 4497.64305317735 4390.80761382767 4285.3349770262 4181.17873682896 4078.2940054479 3976.63734068395 3876.16667713006 3776.84126090677 3678.62158770879 3581.46934395661 3485.34735086099 ...(+2764 chars)]  tireParamSet=vdynPassCar.mat  plySteer=off  turnslip=off  PRESMAX=1000000  PRESMIN=10000  FZMAX=10000  FZMIN=100  VXLOW=0.1  KPUMAX=1.5  KPUMIN=-1.5  ALPMAX=1.5  ALPMIN=-1.5  CAMMAX=0.2  CAMMIN=-0.2  LONGVL=16.7  omegao=0  br=1e-3  UNLOADED_RADIUS=0.42  NOMPRES=224000  FNOMIN=4000  WIDTH=0.209  MASS=9.46+20  IYY=0.740633832792491  GRAVITY=-9.81  zo=.015  zdoto=0  BREFF=8.25094594147963  DREFF=0.260468730454265  FREFF=0.0735298544471851  Q_RE0=1.00866439868088  Q_V1=0.000760413786224011  Q_V2=0.0463384792019201  Q_FZ1=0  Q_FZ2=15.6870832810226  Q_FZ3=0  Q_FCX=0.138643970247602  Q_FCY=0.10843499565426  Q_FCY2=-0.465763352339538  PFZ1=0.69958166705601  VERTICAL_STIFFNESS=207885.061134007  VERTICAL_DAMPING=494.649255786991  LONGITUDINAL_STIFFNESS=388714.175879854  LATERAL_STIFFNESS=157087.404633332  PCFX1=0.18539229191199  PCFX2=0  PCFX3=0  PCFY1=0.163183345037677  PCFY2=0  PCFY3=0.249094918231954  Q_RA1=0.675942571700787  Q_RA2=0.73800463546164  Q_RB1=1.04487486456705  Q_RB2=-1.191763806629  PCX1=1.58523057950359  PDX1=1.0239116238178  PDX2=-0.0842405110022724  PDX3=0  PEX1=0.110312777158455  PEX2=0.313468516038146  PEX3=0  PEX4=0.0016060905760045  PKX1=21.3872544684023  PKX2=14.0006541873175  PKX3=-0.405326109653452  PHX1=0.000212599305364818  PHX2=0.00115950515263055  PVX1=1.59236164471432e-05  PVX2=0.000104321112127671  PPX1=-0.349461321276586  PPX2=0.387840040616429  PPX3=-0.0969947336569324  PPX4=0.0632271859795801  RBX1=12.7633329850276  RBX2=9.5787123658471  RBX3=0  RCX1=1.02796280922059  REX1=-0.45202516851367  REX2=-0.47304886171176  RHX1=0.000233272373115809  QSX1=-0.00788307788961443  QSX2=0.954629515459396  QSX3=0.0155855777667025  QSX4=0.125904607142414  QSX5=1.01110069703963  QSX6=20.1938577118433  QSX7=0.310818120717083  QSX8=-0.0430823751139655  QSX9=0.636494404888216  QSX10=0.142438060591663  QSX11=0.346766530036373  QSX12=0  QSX13=0  QSX14=0  PPMX1=0  PCY1=1.34299950037631  PDY1=0.878267729082195  PDY2=-0.0644597923147385  PDY3=0  PEY1=-0.809776534470972  PEY2=-0.600180598867198  PEY3=0.0991732552633487  PEY4=-6.5577974035573  PEY5=0  PKY1=-15.5714726518315  PKY2=1.73126522291751  PKY3=0.365349873517229  PKY4=1.98176755955416  PKY5=0  PKY6=-0.884005199550313  PKY7=-0.237259727611847  PHY1=-0.00183370557235628  PHY2=0.00346401302716671  PVY1=-0.00675427560163264  PVY2=0.036379218103843  PVY3=-0.163543984089166  PVY4=-0.491003349625726  PPY1=-0.62059646553185  PPY2=-0.0647824842338686  PPY3=-0.164648843290686  PPY4=0.283193909060098  PPY5=0  RBY1=10.7588809173639  RBY2=7.70420065295029  RBY3=3.40283755070691e-06  RBY4=0  RCY1=1.06691874059059  REY1=0.308244924574305  REY2=7.48775032604508e-06  RHY1=0.0118479204960415  RHY2=7.63650177161071e-06  RVY1=0.0560024425050078  RVY2=7.48487127056197e-06  RVY3=0  RVY4=98.4047026517149  RVY5=2.02759273900054  RVY6=15.7623064923347  QSY1=0.00699077564863536  QSY2=0  QSY3=0.00153535478298811  QSY4=8.55710322455322e-05  QSY5=0  QSY6=0  QSY7=0.89443879773793  QSY8=-0.403227641260894  QBZ1=11.666656027484  QBZ2=-1.30355438574485  QBZ3=0  QBZ4=0.177918305399071  QBZ5=-0.162481135068033  QBZ6=0  QBZ9=30.1445534682089  QBZ10=0  QCZ1=1.29026978207574  QDZ1=0.0886972644991399  QDZ2=-0.0058634820161856  QDZ3=0.3805597481383  QDZ4=0  QDZ6=0.00160914918118959  QDZ7=-0.00211036330862154  QDZ8=-0.13921904912557  QDZ9=0.00816585550028243  QDZ10=0  QDZ11=0  QEZ1=-2.19802254534746  QEZ2=1.01850535789165  QEZ3=0  QEZ4=0.278379679112054  QEZ5=-0.548414722765386  QHZ1=0.00148361198869669  QHZ2=0.00202017567585904  QHZ3=0.240316641332066  QHZ4=-0.210114035738085  PPZ1=-0.443927982388615  PPZ2=0  SSZ1=0.00914999585397887  SSZ2=0.0389830656052735  SSZ3=0  SSZ4=0  PDXP1=0.396718274678791  PDXP2=0  PDXP3=0  PKYP1=1.00587060633573  PDYP1=0.40483048923438  PDYP2=0  PDYP3=0  PDYP4=0  PHYP1=0.992731942067188  PHYP2=0.150352945499914  PHYP3=0  PHYP4=-3.98988682633674  PECP1=0.502379254513503  PECP2=0  QDTP1=10.0178654287947  QCRP1=0.200627747200702  QCRP2=0.0995735881599772  QBRP1=0.0997107127960717  QDRP1=1.01432910167423  QDRP2=0  aMode=2
      settings: SourceProductName=Vehicle Dynamics Blockset
  Combined Slip Wheel 2DOF - FrontLeft - TUM : vehdynlibtire_TUM/Combined Slip Wheel 2DOF  BrakeType=Disc  mu_static=VEH__Brakes__mue_BrakePadsFrRe_static__1  mu_kinetic=VEH__Brakes__mue_BrakePadsFrRe_kinetic__1  disk_abore=VEH__Brakes__d_BrakeActuatorBoreFrRe_m__1  Rm=VEH__Brakes__r_BrakePadsMeanLeverFrRe_m__1  num_pads=VEH__Brakes__n_BrakePadsNumberFrRe__1  drum_abore=0.0508  drum_a=0.123  drum_c=0.212  drum_r=0.15  drum_theta1=0  drum_theta2=126  brake_p_bpt=[1 11.4736842105263 21.9473684210526 32.4210526315789 42.8947368421053 53.3684210526316 63.8421052631579 74.3157894736842 84.7894736842105 95.2631578947368 105.736842105263 116.210526315789 126.684210526316 137.157894736842 147.631578947368 158.105263157895 168.578947368421 179.052631578947 189.526315789474 200]  brake_n_bpt=[0 52.6315789473684 105.263157894737 157.894736842105 210.526315789474 263.157894736842 315.789473684211 368.421052631579 421.052631578947 473.684210526316 526.315789473684 578.947368421053 631.578947368421 684.210526315789 736.842105263158 789.473684210526 842.105263157895 894.736842105263 947.368421052632 1000]  f_brake_t=[43.4900602404453 42.5056030554862 41.5350898940194 40.5780454442085 39.6340111501808 38.7025443887544 37.7832176914519 36.8756180088306 35.9793460143796 35.0940154454303 34.2192524787115 33.3546951383474 32.4999927342521 31.6548053290159 30.8188032315107 29.991666515561 29.1730845621415 28.362755623661 27.5603864089927 26.765691687993;498.991217495636 487.695866636631 476.560505099801 465.579679307235 454.748127933653 444.060772460445 433.51270824929 423.099196101319 412.81565427025 402.657650900201 392.620896861006 382.701238955775 372.894653477208 363.197240090814 353.605216024701 344.114910546964 334.722759712992 325.425301366216 316.219170376863 307.10109410434;954.492374750826 932.886130217776 911.585920305583 890.581313170261 869.862244717126 849.419000532136 829.242198807128 809.322774193808 789.651962526121 770.221286354971 751.0225412433 732.047782773203 713.289314220164 694.739674852612 676.391628817892 658.238154578366 640.272434863842 622.48784710877 604.877954344734 587.436496520688;1409.99353200602 1378.07639379892 1346.61133551136 1315.58294703329 1284.9763615006 1254.77722860383 1224.97168936497 1195.5463522863 1166.48827078199 1137.78492180974 1109.42418562559 1081.39432659063 1053.68397496312 1026.28210961441 999.178041611083 972.361398609768 945.822110014692 919.550392851325 893.536738312604 867.771898937035;1865.49468926121 1823.26665738007 1781.63675071715 1740.58458089631 1700.09047828407 1660.13545667552 1620.7011799228 1581.76993037878 1543.32457903786 1505.34855726451 1467.82583000789 1430.74087040806 1394.07863570608 1357.82454437621 1321.96445440427 1286.48464264117 1251.37178516554 1216.61293859388 1182.19552228048 1148.10730135338;2320.9958465164 2268.45692096121 2216.66216592293 2165.58621475934 2115.20459506754 2065.49368474721 2016.43067048064 1967.99350847127 1920.16088729373 1872.91219271928 1826.22747439018 1780.08741422549 1734.47329644903 1689.36697913801 1644.75086719747 1600.60788667257 1556.92146031639 1513.67548433643 1470.85430624835 1428.44270376973;2776.49700377159 2713.64718454235 2651.68758112871 2590.58784862237 2530.31871185102 2470.8519128189 2412.16016103848 2354.21708656376 2296.9971955496 2240.47582817405 2184.62911877248 2129.43395804292 2074.86795719199 2020.9094138998 1967.53727999066 1914.73113070398 1862.47113546724 1810.73803007899 1759.51309021622 1708.77810618608;3231.99816102678 3158.8374481235 3086.71299633449 3015.58948248539 2945.43282863449 2876.21014089059 2807.88965159632 2740.44066465625 2673.83350380547 2608.03946362882 2543.03076315477 2478.78050186034 2415.26261793494 2352.4518486616 2290.32369278385 2228.85437473538 2168.02081061809 2107.80057582154 2048.17187418409 1989.11350860242;3687.49931828197 3604.02771170464 3521.73841154027 3440.59111634842 3360.54694541796 3281.56836896228 3203.61914215416 3126.66424274874 3050.66981206134 2975.60309908359 2901.43240753707 2828.12704567777 2755.6572786779 2683.9942834234 2613.11010557704 2542.97761876678 2473.57048576894 2404.8631215641 2336.83065815196 2269.44891101877;4143.00047553716 4049.21797528579 3956.76382674606 3865.59275021144 3775.66106220143 3686.92659703397 3599.34863271199 3512.88782084123 3427.50612031721 3343.16673453836 3259.83405191936 3177.4735894952 3096.05193942085 3015.5367181852 2935.89651837023 2857.10086279818 2779.12016091979 2701.92566730665 2625.48944211983 2549.78431343512;4598.50163279235 4494.40823886693 4391.78924195184 4290.59438407447 4190.77517898491 4092.28482510566 3995.07812326983 3899.11139893372 3804.34242857308 3710.73036999313 3618.23569630166 3526.82013331263 3436.44660016381 3347.079152947 3258.68293116342 3171.22410682959 3084.66983607064 2998.98821304921 2914.1482260877 2830.11971585147;5054.00279004754 4939.59850244808 4826.81465715762 4715.59601793749 4605.88929576838 4497.64305317735 4390.80761382767 4285.3349770262 4181.17873682896 4078.2940054479 3976.63734068395 3876.16667713006 3776.84126090677 3678.62158770879 3581.46934395661 3485.34735086099 ...(+2764 chars)]  tireParamSet=vdynPassCar.mat  plySteer=off  turnslip=off  PRESMAX=tireFL__SIMULATION__PRESMAX  PRESMIN=tireFL__SIMULATION__PRESMIN  FZMAX=tireFL__SIMULATION__FZMAX  FZMIN=tireFL__SIMULATION__FZMIN  VXLOW=tireFL__SIMULATION__VXLOW  KPUMAX=tireFL__SIMULATION__KPUMAX  KPUMIN=tireFL__SIMULATION__KPUMIN  ALPMAX=tireFL__SIMULATION__ALPMAX  ALPMIN=tireFL__SIMULATION__ALPMIN  CAMMAX=tireFL__SIMULATION__CAMMAX  CAMMIN=tireFL__SIMULATION__CAMMIN  LONGVL=tireFL__SIMULATION__LONGVL  omegao=INIT__initialvalues__omega0_Wheels_radps__1  br=tireFL__WHEEL__br_Nmsprad  UNLOADED_RADIUS=tireFL__WHEEL__TYRE_RADIUS_MOD  NOMPRES=tireFL__WHEEL__NORMPRES  FNOMIN=tireFL__WHEEL__FNOMIN  WIDTH=tireFL__DIMENSION__WIDTH  MASS=tireFL__INERTIAL__m_Wheel_kg  IYY=tireFL__INERTIAL__Iyy_Wheel_kgm2  GRAVITY=- VEH__Environment__a_Gravity_mps2  zo=INIT__initialvalues__z0_TireDeflection_m__1  zdoto=INIT__initialvalues__v0z_Wheels_mps__1  BREFF=tireFL__VERTICAL__BREFF  DREFF=tireFL__VERTICAL__DREFF  FREFF=tireFL__VERTICAL__FREFF  Q_RE0=tireFL__VERTICAL__Q_RE0  Q_V1=tireFL__VERTICAL__Q_V1  Q_V2=tireFL__VERTICAL__Q_V2  Q_FZ1=tireFL__VERTICAL__Q_FZ1  Q_FZ2=tireFL__VERTICAL__Q_FZ2  Q_FZ3=tireFL__VERTICAL__Q_FZ3  Q_FCX=tireFL__VERTICAL__Q_FCX  Q_FCY=tireFL__VERTICAL__Q_FCY  Q_FCY2=tireFL__VERTICAL__Q_FCY2  PFZ1=tireFL__VERTICAL__PFZ1  VERTICAL_STIFFNESS=tireFL__VERTICAL__VERTICAL_STIFFNESS  VERTICAL_DAMPING=tireFL__VERTICAL__VERTICAL_DAMPING  LONGITUDINAL_STIFFNESS=tireFL__STRUCTURAL__LONGITUDINAL_STIFFNESS  LATERAL_STIFFNESS=tireFL__STRUCTURAL__LATERAL_STIFFNESS  PCFX1=tireFL__STRUCTURAL__PCFX1  PCFX2=tireFL__STRUCTURAL__PCFX2  PCFX3=tireFL__STRUCTURAL__PCFX3  PCFY1=tireFL__STRUCTURAL__PCFY1  PCFY2=tireFL__STRUCTURAL__PCFY2  PCFY3=tireFL__STRUCTURAL__PCFY3  Q_RA1=tireFL__CONTACTPATCH__Q_RA1  Q_RA2=tireFL__CONTACTPATCH__Q_RA2  Q_RB1=tireFL__CONTACTPATCH__Q_RB1  Q_RB2=tireFL__CONTACTPATCH__Q_RB2  PCX1=tireFL__LONGITUDINAL__PCX1  PDX1=tireFL__LONGITUDINAL__PDX1  PDX2=tireFL__LONGITUDINAL__PDX2  PDX3=tireFL__LONGITUDINAL__PDX3  PEX1=tireFL__LONGITUDINAL__PEX1  PEX2=tireFL__LONGITUDINAL__PEX2  PEX3=tireFL__LONGITUDINAL__PEX3  PEX4=tireFL__LONGITUDINAL__PEX4  PKX1=tireFL__LONGITUDINAL__PKX1  PKX2=tireFL__LONGITUDINAL__PKX2  PKX3=tireFL__LONGITUDINAL__PKX3  PHX1=tireFL__LONGITUDINAL__PHX1  PHX2=tireFL__LONGITUDINAL__PHX2  PVX1=tireFL__LONGITUDINAL__PVX1  PVX2=tireFL__LONGITUDINAL__PVX2  PPX1=tireFL__LONGITUDINAL__PPX1  PPX2=tireFL__LONGITUDINAL__PPX2  PPX3=tireFL__LONGITUDINAL__PPX3  PPX4=tireFL__LONGITUDINAL__PPX4  RBX1=tireFL__LONGITUDINAL__RBX1  RBX2=tireFL__LONGITUDINAL__RBX2  RBX3=tireFL__LONGITUDINAL__RBX3  RCX1=tireFL__LONGITUDINAL__RCX1  REX1=tireFL__LONGITUDINAL__REX1  REX2=tireFL__LONGITUDINAL__REX2  RHX1=tireFL__LONGITUDINAL__RHX1  QSX1=tireFL__OVERTURNING__QSX1  QSX2=tireFL__OVERTURNING__QSX2  QSX3=tireFL__OVERTURNING__QSX3  QSX4=tireFL__OVERTURNING__QSX4  QSX5=tireFL__OVERTURNING__QSX5  QSX6=tireFL__OVERTURNING__QSX6  QSX7=tireFL__OVERTURNING__QSX7  QSX8=tireFL__OVERTURNING__QSX8  QSX9=tireFL__OVERTURNING__QSX9  QSX10=tireFL__OVERTURNING__QSX10  QSX11=tireFL__OVERTURNING__QSX11  QSX12=tireFL__OVERTURNING__QSX12  QSX13=tireFL__OVERTURNING__QSX13  QSX14=tireFL__OVERTURNING__QSX14  PPMX1=tireFL__OVERTURNING__PPMX1  PCY1=tireFL__LATERAL__PCY1  PDY1=tireFL__LATERAL__PDY1  PDY2=tireFL__LATERAL__PDY2  PDY3=tireFL__LATERAL__PDY3  PEY1=tireFL__LATERAL__PEY1  PEY2=tireFL__LATERAL__PEY2  PEY3=tireFL__LATERAL__PEY3  PEY4=tireFL__LATERAL__PEY4  PEY5=tireFL__LATERAL__PEY5  PKY1=tireFL__LATERAL__PKY1  PKY2=tireFL__LATERAL__PKY2  PKY3=tireFL__LATERAL__PKY3  PKY4=tireFL__LATERAL__PKY4  PKY5=tireFL__LATERAL__PKY5  PKY6=tireFL__LATERAL__PKY6  PKY7=tireFL__LATERAL__PKY7  PHY1=tireFL__LATERAL__PHY1  PHY2=tireFL__LATERAL__PHY2  PVY1=tireFL__LATERAL__PVY1  PVY2=tireFL__LATERAL__PVY2  PVY3=tireFL__LATERAL__PVY3  PVY4=tireFL__LATERAL__PVY4  PPY1=tireFL__LATERAL__PPY1  PPY2=tireFL__LATERAL__PPY2  PPY3=tireFL__LATERAL__PPY3  PPY4=tireFL__LATERAL__PPY4  PPY5=tireFL__LATERAL__PPY5  RBY1=tireFL__LATERAL__RBY1  RBY2=tireFL__LATERAL__RBY2  RBY3=tireFL__LATERAL__RBY3  RBY4=tireFL__LATERAL__RBY4  RCY1=tireFL__LATERAL__RCY1  REY1=tireFL__LATERAL__REY1  REY2=tireFL__LATERAL__REY2  RHY1=tireFL__LATERAL__RHY1  RHY2=tireFL__LATERAL__RHY2  RVY1=tireFL__LATERAL__RVY1  RVY2=tireFL__LATERAL__RVY2  RVY3=tireFL__LATERAL__RVY3  RVY4=tireFL__LATERAL__RVY4  RVY5=tireFL__LATERAL__RVY5  RVY6=tireFL__LATERAL__RVY6  QSY1=tireFL__ROLLING__QSY1  QSY2=tireFL__ROLLING__QSY2  QSY3=tireFL__ROLLING__QSY3  QSY4=tireFL__ROLLING__QSY4  QSY5=tireFL__ROLLING__QSY5  QSY6=tireFL__ROLLING__QSY6  QSY7=tireFL__ROLLING__QSY7  QSY8=tireFL__ROLLING__QSY8  QBZ1=tireFL__ALIGNING__QBZ1  QBZ2=tireFL__ALIGNING__QBZ2  QBZ3=tireFL__ALIGNING__QBZ3  QBZ4=tireFL__ALIGNING__QBZ4  QBZ5=tireFL__ALIGNING__QBZ5  QBZ6=tireFL__ALIGNING__QBZ6  QBZ9=tireFL__ALIGNING__QBZ9  QBZ10=tireFL__ALIGNING__QBZ10  QCZ1=tireFL__ALIGNING__QCZ1  QDZ1=tireFL__ALIGNING__QDZ1  QDZ2=tireFL__ALIGNING__QDZ2  QDZ3=tireFL__ALIGNING__QDZ3  QDZ4=tireFL__ALIGNING__QDZ4  QDZ6=tireFL__ALIGNING__QDZ6  QDZ7=tireFL__ALIGNING__QDZ7  QDZ8=tireFL__ALIGNING__QDZ8  QDZ9=tireFL__ALIGNING__QDZ9  QDZ10=tireFL__ALIGNING__QDZ10  QDZ11=tireFL__ALIGNING__QDZ11  QEZ1=tireFL__ALIGNING__QEZ1  QEZ2=tireFL__ALIGNING__QEZ2  QEZ3=tireFL__ALIGNING__QEZ3  QEZ4=tireFL__ALIGNING__QEZ4  QEZ5=tireFL__ALIGNING__QEZ5  QHZ1=tireFL__ALIGNING__QHZ1  QHZ2=tireFL__ALIGNING__QHZ2  QHZ3=tireFL__ALIGNING__QHZ3  QHZ4=tireFL__ALIGNING__QHZ4  PPZ1=tireFL__ALIGNING__PPZ1  PPZ2=tireFL__ALIGNING__PPZ2  SSZ1=tireFL__ALIGNING__SSZ1  SSZ2=tireFL__ALIGNING__SSZ2  SSZ3=tireFL__ALIGNING__SSZ3  SSZ4=tireFL__ALIGNING__SSZ4  PDXP1=tireFL__TURNSLIP__PDXP1  PDXP2=tireFL__TURNSLIP__PDXP2  PDXP3=tireFL__TURNSLIP__PDXP3  PKYP1=tireFL__TURNSLIP__PKYP1  PDYP1=tireFL__TURNSLIP__PDYP1  PDYP2=tireFL__TURNSLIP__PDYP2  PDYP3=tireFL__TURNSLIP__PDYP3  PDYP4=tireFL__TURNSLIP__PDYP4  PHYP1=tireFL__TURNSLIP__PHYP1  PHYP2=tireFL__TURNSLIP__PHYP2  PHYP3=tireFL__TURNSLIP__PHYP3  PHYP4=tireFL__TURNSLIP__PHYP4  PECP1=tireFL__TURNSLIP__PECP1  PECP2=tireFL__TURNSLIP__PECP2  QDTP1=tireFL__TURNSLIP__QDTP1  QCRP1=tireFL__TURNSLIP__QCRP1  QCRP2=tireFL__TURNSLIP__QCRP2  QBRP1=tireFL__TURNSLIP__QBRP1  QDRP1=tireFL__TURNSLIP__QDRP1  QDRP2=tireFL__TURNSLIP__QDRP2  aMode=2
  Combined Slip Wheel 2DOF - FrontRight - TUM : vehdynlibtire_TUM/Combined Slip Wheel 2DOF  BrakeType=Disc  mu_static=VEH__Brakes__mue_BrakePadsFrRe_static__1  mu_kinetic=VEH__Brakes__mue_BrakePadsFrRe_kinetic__1  disk_abore=VEH__Brakes__d_BrakeActuatorBoreFrRe_m__1  Rm=VEH__Brakes__r_BrakePadsMeanLeverFrRe_m__1  num_pads=VEH__Brakes__n_BrakePadsNumberFrRe__1  drum_abore=0.0508  drum_a=0.123  drum_c=0.212  drum_r=0.15  drum_theta1=0  drum_theta2=126  brake_p_bpt=[1 11.4736842105263 21.9473684210526 32.4210526315789 42.8947368421053 53.3684210526316 63.8421052631579 74.3157894736842 84.7894736842105 95.2631578947368 105.736842105263 116.210526315789 126.684210526316 137.157894736842 147.631578947368 158.105263157895 168.578947368421 179.052631578947 189.526315789474 200]  brake_n_bpt=[0 52.6315789473684 105.263157894737 157.894736842105 210.526315789474 263.157894736842 315.789473684211 368.421052631579 421.052631578947 473.684210526316 526.315789473684 578.947368421053 631.578947368421 684.210526315789 736.842105263158 789.473684210526 842.105263157895 894.736842105263 947.368421052632 1000]  f_brake_t=[43.4900602404453 42.5056030554862 41.5350898940194 40.5780454442085 39.6340111501808 38.7025443887544 37.7832176914519 36.8756180088306 35.9793460143796 35.0940154454303 34.2192524787115 33.3546951383474 32.4999927342521 31.6548053290159 30.8188032315107 29.991666515561 29.1730845621415 28.362755623661 27.5603864089927 26.765691687993;498.991217495636 487.695866636631 476.560505099801 465.579679307235 454.748127933653 444.060772460445 433.51270824929 423.099196101319 412.81565427025 402.657650900201 392.620896861006 382.701238955775 372.894653477208 363.197240090814 353.605216024701 344.114910546964 334.722759712992 325.425301366216 316.219170376863 307.10109410434;954.492374750826 932.886130217776 911.585920305583 890.581313170261 869.862244717126 849.419000532136 829.242198807128 809.322774193808 789.651962526121 770.221286354971 751.0225412433 732.047782773203 713.289314220164 694.739674852612 676.391628817892 658.238154578366 640.272434863842 622.48784710877 604.877954344734 587.436496520688;1409.99353200602 1378.07639379892 1346.61133551136 1315.58294703329 1284.9763615006 1254.77722860383 1224.97168936497 1195.5463522863 1166.48827078199 1137.78492180974 1109.42418562559 1081.39432659063 1053.68397496312 1026.28210961441 999.178041611083 972.361398609768 945.822110014692 919.550392851325 893.536738312604 867.771898937035;1865.49468926121 1823.26665738007 1781.63675071715 1740.58458089631 1700.09047828407 1660.13545667552 1620.7011799228 1581.76993037878 1543.32457903786 1505.34855726451 1467.82583000789 1430.74087040806 1394.07863570608 1357.82454437621 1321.96445440427 1286.48464264117 1251.37178516554 1216.61293859388 1182.19552228048 1148.10730135338;2320.9958465164 2268.45692096121 2216.66216592293 2165.58621475934 2115.20459506754 2065.49368474721 2016.43067048064 1967.99350847127 1920.16088729373 1872.91219271928 1826.22747439018 1780.08741422549 1734.47329644903 1689.36697913801 1644.75086719747 1600.60788667257 1556.92146031639 1513.67548433643 1470.85430624835 1428.44270376973;2776.49700377159 2713.64718454235 2651.68758112871 2590.58784862237 2530.31871185102 2470.8519128189 2412.16016103848 2354.21708656376 2296.9971955496 2240.47582817405 2184.62911877248 2129.43395804292 2074.86795719199 2020.9094138998 1967.53727999066 1914.73113070398 1862.47113546724 1810.73803007899 1759.51309021622 1708.77810618608;3231.99816102678 3158.8374481235 3086.71299633449 3015.58948248539 2945.43282863449 2876.21014089059 2807.88965159632 2740.44066465625 2673.83350380547 2608.03946362882 2543.03076315477 2478.78050186034 2415.26261793494 2352.4518486616 2290.32369278385 2228.85437473538 2168.02081061809 2107.80057582154 2048.17187418409 1989.11350860242;3687.49931828197 3604.02771170464 3521.73841154027 3440.59111634842 3360.54694541796 3281.56836896228 3203.61914215416 3126.66424274874 3050.66981206134 2975.60309908359 2901.43240753707 2828.12704567777 2755.6572786779 2683.9942834234 2613.11010557704 2542.97761876678 2473.57048576894 2404.8631215641 2336.83065815196 2269.44891101877;4143.00047553716 4049.21797528579 3956.76382674606 3865.59275021144 3775.66106220143 3686.92659703397 3599.34863271199 3512.88782084123 3427.50612031721 3343.16673453836 3259.83405191936 3177.4735894952 3096.05193942085 3015.5367181852 2935.89651837023 2857.10086279818 2779.12016091979 2701.92566730665 2625.48944211983 2549.78431343512;4598.50163279235 4494.40823886693 4391.78924195184 4290.59438407447 4190.77517898491 4092.28482510566 3995.07812326983 3899.11139893372 3804.34242857308 3710.73036999313 3618.23569630166 3526.82013331263 3436.44660016381 3347.079152947 3258.68293116342 3171.22410682959 3084.66983607064 2998.98821304921 2914.1482260877 2830.11971585147;5054.00279004754 4939.59850244808 4826.81465715762 4715.59601793749 4605.88929576838 4497.64305317735 4390.80761382767 4285.3349770262 4181.17873682896 4078.2940054479 3976.63734068395 3876.16667713006 3776.84126090677 3678.62158770879 3581.46934395661 3485.34735086099 ...(+2764 chars)]  tireParamSet=vdynPassCar.mat  plySteer=off  turnslip=off  PRESMAX=tireFR__SIMULATION__PRESMAX  PRESMIN=tireFR__SIMULATION__PRESMIN  FZMAX=tireFR__SIMULATION__FZMAX  FZMIN=tireFR__SIMULATION__FZMIN  VXLOW=tireFR__SIMULATION__VXLOW  KPUMAX=tireFR__SIMULATION__KPUMAX  KPUMIN=tireFR__SIMULATION__KPUMIN  ALPMAX=tireFR__SIMULATION__ALPMAX  ALPMIN=tireFR__SIMULATION__ALPMIN  CAMMAX=tireFR__SIMULATION__CAMMAX  CAMMIN=tireFR__SIMULATION__CAMMIN  LONGVL=tireFR__SIMULATION__LONGVL  omegao=INIT__initialvalues__omega0_Wheels_radps__2  br=tireFR__WHEEL__br_Nmsprad  UNLOADED_RADIUS=tireFR__WHEEL__TYRE_RADIUS_MOD  NOMPRES=tireFR__WHEEL__NORMPRES  FNOMIN=tireFR__WHEEL__FNOMIN  WIDTH=tireFR__DIMENSION__WIDTH  MASS=tireFR__INERTIAL__m_Wheel_kg  IYY=tireFR__INERTIAL__Iyy_Wheel_kgm2  GRAVITY=- VEH__Environment__a_Gravity_mps2  zo=INIT__initialvalues__z0_TireDeflection_m__2  zdoto=INIT__initialvalues__v0z_Wheels_mps__2  BREFF=tireFR__VERTICAL__BREFF  DREFF=tireFR__VERTICAL__DREFF  FREFF=tireFR__VERTICAL__FREFF  Q_RE0=tireFR__VERTICAL__Q_RE0  Q_V1=tireFR__VERTICAL__Q_V1  Q_V2=tireFR__VERTICAL__Q_V2  Q_FZ1=tireFR__VERTICAL__Q_FZ1  Q_FZ2=tireFR__VERTICAL__Q_FZ2  Q_FZ3=tireFR__VERTICAL__Q_FZ3  Q_FCX=tireFR__VERTICAL__Q_FCX  Q_FCY=tireFR__VERTICAL__Q_FCY  Q_FCY2=tireFR__VERTICAL__Q_FCY2  PFZ1=tireFR__VERTICAL__PFZ1  VERTICAL_STIFFNESS=tireFR__VERTICAL__VERTICAL_STIFFNESS  VERTICAL_DAMPING=tireFR__VERTICAL__VERTICAL_DAMPING  LONGITUDINAL_STIFFNESS=tireFR__STRUCTURAL__LONGITUDINAL_STIFFNESS  LATERAL_STIFFNESS=tireFR__STRUCTURAL__LATERAL_STIFFNESS  PCFX1=tireFR__STRUCTURAL__PCFX1  PCFX2=tireFR__STRUCTURAL__PCFX2  PCFX3=tireFR__STRUCTURAL__PCFX3  PCFY1=tireFR__STRUCTURAL__PCFY1  PCFY2=tireFR__STRUCTURAL__PCFY2  PCFY3=tireFR__STRUCTURAL__PCFY3  Q_RA1=tireFR__CONTACTPATCH__Q_RA1  Q_RA2=tireFR__CONTACTPATCH__Q_RA2  Q_RB1=tireFR__CONTACTPATCH__Q_RB1  Q_RB2=tireFR__CONTACTPATCH__Q_RB2  PCX1=tireFR__LONGITUDINAL__PCX1  PDX1=tireFR__LONGITUDINAL__PDX1  PDX2=tireFR__LONGITUDINAL__PDX2  PDX3=tireFR__LONGITUDINAL__PDX3  PEX1=tireFR__LONGITUDINAL__PEX1  PEX2=tireFR__LONGITUDINAL__PEX2  PEX3=tireFR__LONGITUDINAL__PEX3  PEX4=tireFR__LONGITUDINAL__PEX4  PKX1=tireFR__LONGITUDINAL__PKX1  PKX2=tireFR__LONGITUDINAL__PKX2  PKX3=tireFR__LONGITUDINAL__PKX3  PHX1=tireFR__LONGITUDINAL__PHX1  PHX2=tireFR__LONGITUDINAL__PHX2  PVX1=tireFR__LONGITUDINAL__PVX1  PVX2=tireFR__LONGITUDINAL__PVX2  PPX1=tireFR__LONGITUDINAL__PPX1  PPX2=tireFR__LONGITUDINAL__PPX2  PPX3=tireFR__LONGITUDINAL__PPX3  PPX4=tireFR__LONGITUDINAL__PPX4  RBX1=tireFR__LONGITUDINAL__RBX1  RBX2=tireFR__LONGITUDINAL__RBX2  RBX3=tireFR__LONGITUDINAL__RBX3  RCX1=tireFR__LONGITUDINAL__RCX1  REX1=tireFR__LONGITUDINAL__REX1  REX2=tireFR__LONGITUDINAL__REX2  RHX1=tireFR__LONGITUDINAL__RHX1  QSX1=tireFR__OVERTURNING__QSX1  QSX2=tireFR__OVERTURNING__QSX2  QSX3=tireFR__OVERTURNING__QSX3  QSX4=tireFR__OVERTURNING__QSX4  QSX5=tireFR__OVERTURNING__QSX5  QSX6=tireFR__OVERTURNING__QSX6  QSX7=tireFR__OVERTURNING__QSX7  QSX8=tireFR__OVERTURNING__QSX8  QSX9=tireFR__OVERTURNING__QSX9  QSX10=tireFR__OVERTURNING__QSX10  QSX11=tireFR__OVERTURNING__QSX11  QSX12=tireFR__OVERTURNING__QSX12  QSX13=tireFR__OVERTURNING__QSX13  QSX14=tireFR__OVERTURNING__QSX14  PPMX1=tireFR__OVERTURNING__PPMX1  PCY1=tireFR__LATERAL__PCY1  PDY1=tireFR__LATERAL__PDY1  PDY2=tireFR__LATERAL__PDY2  PDY3=tireFR__LATERAL__PDY3  PEY1=tireFR__LATERAL__PEY1  PEY2=tireFR__LATERAL__PEY2  PEY3=tireFR__LATERAL__PEY3  PEY4=tireFR__LATERAL__PEY4  PEY5=tireFR__LATERAL__PEY5  PKY1=tireFR__LATERAL__PKY1  PKY2=tireFR__LATERAL__PKY2  PKY3=tireFR__LATERAL__PKY3  PKY4=tireFR__LATERAL__PKY4  PKY5=tireFR__LATERAL__PKY5  PKY6=tireFR__LATERAL__PKY6  PKY7=tireFR__LATERAL__PKY7  PHY1=tireFR__LATERAL__PHY1  PHY2=tireFR__LATERAL__PHY2  PVY1=tireFR__LATERAL__PVY1  PVY2=tireFR__LATERAL__PVY2  PVY3=tireFR__LATERAL__PVY3  PVY4=tireFR__LATERAL__PVY4  PPY1=tireFR__LATERAL__PPY1  PPY2=tireFR__LATERAL__PPY2  PPY3=tireFR__LATERAL__PPY3  PPY4=tireFR__LATERAL__PPY4  PPY5=tireFR__LATERAL__PPY5  RBY1=tireFR__LATERAL__RBY1  RBY2=tireFR__LATERAL__RBY2  RBY3=tireFR__LATERAL__RBY3  RBY4=tireFR__LATERAL__RBY4  RCY1=tireFR__LATERAL__RCY1  REY1=tireFR__LATERAL__REY1  REY2=tireFR__LATERAL__REY2  RHY1=tireFR__LATERAL__RHY1  RHY2=tireFR__LATERAL__RHY2  RVY1=tireFR__LATERAL__RVY1  RVY2=tireFR__LATERAL__RVY2  RVY3=tireFR__LATERAL__RVY3  RVY4=tireFR__LATERAL__RVY4  RVY5=tireFR__LATERAL__RVY5  RVY6=tireFR__LATERAL__RVY6  QSY1=tireFR__ROLLING__QSY1  QSY2=tireFR__ROLLING__QSY2  QSY3=tireFR__ROLLING__QSY3  QSY4=tireFR__ROLLING__QSY4  QSY5=tireFR__ROLLING__QSY5  QSY6=tireFR__ROLLING__QSY6  QSY7=tireFR__ROLLING__QSY7  QSY8=tireFR__ROLLING__QSY8  QBZ1=tireFR__ALIGNING__QBZ1  QBZ2=tireFR__ALIGNING__QBZ2  QBZ3=tireFR__ALIGNING__QBZ3  QBZ4=tireFR__ALIGNING__QBZ4  QBZ5=tireFR__ALIGNING__QBZ5  QBZ6=tireFR__ALIGNING__QBZ6  QBZ9=tireFR__ALIGNING__QBZ9  QBZ10=tireFR__ALIGNING__QBZ10  QCZ1=tireFR__ALIGNING__QCZ1  QDZ1=tireFR__ALIGNING__QDZ1  QDZ2=tireFR__ALIGNING__QDZ2  QDZ3=tireFR__ALIGNING__QDZ3  QDZ4=tireFR__ALIGNING__QDZ4  QDZ6=tireFR__ALIGNING__QDZ6  QDZ7=tireFR__ALIGNING__QDZ7  QDZ8=tireFR__ALIGNING__QDZ8  QDZ9=tireFR__ALIGNING__QDZ9  QDZ10=tireFR__ALIGNING__QDZ10  QDZ11=tireFR__ALIGNING__QDZ11  QEZ1=tireFR__ALIGNING__QEZ1  QEZ2=tireFR__ALIGNING__QEZ2  QEZ3=tireFR__ALIGNING__QEZ3  QEZ4=tireFR__ALIGNING__QEZ4  QEZ5=tireFR__ALIGNING__QEZ5  QHZ1=tireFR__ALIGNING__QHZ1  QHZ2=tireFR__ALIGNING__QHZ2  QHZ3=tireFR__ALIGNING__QHZ3  QHZ4=tireFR__ALIGNING__QHZ4  PPZ1=tireFR__ALIGNING__PPZ1  PPZ2=tireFR__ALIGNING__PPZ2  SSZ1=tireFR__ALIGNING__SSZ1  SSZ2=tireFR__ALIGNING__SSZ2  SSZ3=tireFR__ALIGNING__SSZ3  SSZ4=tireFR__ALIGNING__SSZ4  PDXP1=tireFR__TURNSLIP__PDXP1  PDXP2=tireFR__TURNSLIP__PDXP2  PDXP3=tireFR__TURNSLIP__PDXP3  PKYP1=tireFR__TURNSLIP__PKYP1  PDYP1=tireFR__TURNSLIP__PDYP1  PDYP2=tireFR__TURNSLIP__PDYP2  PDYP3=tireFR__TURNSLIP__PDYP3  PDYP4=tireFR__TURNSLIP__PDYP4  PHYP1=tireFR__TURNSLIP__PHYP1  PHYP2=tireFR__TURNSLIP__PHYP2  PHYP3=tireFR__TURNSLIP__PHYP3  PHYP4=tireFR__TURNSLIP__PHYP4  PECP1=tireFR__TURNSLIP__PECP1  PECP2=tireFR__TURNSLIP__PECP2  QDTP1=tireFR__TURNSLIP__QDTP1  QCRP1=tireFR__TURNSLIP__QCRP1  QCRP2=tireFR__TURNSLIP__QCRP2  QBRP1=tireFR__TURNSLIP__QBRP1  QDRP1=tireFR__TURNSLIP__QDRP1  QDRP2=tireFR__TURNSLIP__QDRP2  aMode=2
  Combined Slip Wheel 2DOF - RearLeft - TUM : vehdynlibtire_TUM/Combined Slip Wheel 2DOF  BrakeType=Disc  mu_static=VEH__Brakes__mue_BrakePadsFrRe_static__2  mu_kinetic=VEH__Brakes__mue_BrakePadsFrRe_kinetic__2  disk_abore=VEH__Brakes__d_BrakeActuatorBoreFrRe_m__2  Rm=VEH__Brakes__r_BrakePadsMeanLeverFrRe_m__2  num_pads=VEH__Brakes__n_BrakePadsNumberFrRe__2  drum_abore=0.0508  drum_a=0.123  drum_c=0.212  drum_r=0.15  drum_theta1=0  drum_theta2=126  brake_p_bpt=[1 11.4736842105263 21.9473684210526 32.4210526315789 42.8947368421053 53.3684210526316 63.8421052631579 74.3157894736842 84.7894736842105 95.2631578947368 105.736842105263 116.210526315789 126.684210526316 137.157894736842 147.631578947368 158.105263157895 168.578947368421 179.052631578947 189.526315789474 200]  brake_n_bpt=[0 52.6315789473684 105.263157894737 157.894736842105 210.526315789474 263.157894736842 315.789473684211 368.421052631579 421.052631578947 473.684210526316 526.315789473684 578.947368421053 631.578947368421 684.210526315789 736.842105263158 789.473684210526 842.105263157895 894.736842105263 947.368421052632 1000]  f_brake_t=[43.4900602404453 42.5056030554862 41.5350898940194 40.5780454442085 39.6340111501808 38.7025443887544 37.7832176914519 36.8756180088306 35.9793460143796 35.0940154454303 34.2192524787115 33.3546951383474 32.4999927342521 31.6548053290159 30.8188032315107 29.991666515561 29.1730845621415 28.362755623661 27.5603864089927 26.765691687993;498.991217495636 487.695866636631 476.560505099801 465.579679307235 454.748127933653 444.060772460445 433.51270824929 423.099196101319 412.81565427025 402.657650900201 392.620896861006 382.701238955775 372.894653477208 363.197240090814 353.605216024701 344.114910546964 334.722759712992 325.425301366216 316.219170376863 307.10109410434;954.492374750826 932.886130217776 911.585920305583 890.581313170261 869.862244717126 849.419000532136 829.242198807128 809.322774193808 789.651962526121 770.221286354971 751.0225412433 732.047782773203 713.289314220164 694.739674852612 676.391628817892 658.238154578366 640.272434863842 622.48784710877 604.877954344734 587.436496520688;1409.99353200602 1378.07639379892 1346.61133551136 1315.58294703329 1284.9763615006 1254.77722860383 1224.97168936497 1195.5463522863 1166.48827078199 1137.78492180974 1109.42418562559 1081.39432659063 1053.68397496312 1026.28210961441 999.178041611083 972.361398609768 945.822110014692 919.550392851325 893.536738312604 867.771898937035;1865.49468926121 1823.26665738007 1781.63675071715 1740.58458089631 1700.09047828407 1660.13545667552 1620.7011799228 1581.76993037878 1543.32457903786 1505.34855726451 1467.82583000789 1430.74087040806 1394.07863570608 1357.82454437621 1321.96445440427 1286.48464264117 1251.37178516554 1216.61293859388 1182.19552228048 1148.10730135338;2320.9958465164 2268.45692096121 2216.66216592293 2165.58621475934 2115.20459506754 2065.49368474721 2016.43067048064 1967.99350847127 1920.16088729373 1872.91219271928 1826.22747439018 1780.08741422549 1734.47329644903 1689.36697913801 1644.75086719747 1600.60788667257 1556.92146031639 1513.67548433643 1470.85430624835 1428.44270376973;2776.49700377159 2713.64718454235 2651.68758112871 2590.58784862237 2530.31871185102 2470.8519128189 2412.16016103848 2354.21708656376 2296.9971955496 2240.47582817405 2184.62911877248 2129.43395804292 2074.86795719199 2020.9094138998 1967.53727999066 1914.73113070398 1862.47113546724 1810.73803007899 1759.51309021622 1708.77810618608;3231.99816102678 3158.8374481235 3086.71299633449 3015.58948248539 2945.43282863449 2876.21014089059 2807.88965159632 2740.44066465625 2673.83350380547 2608.03946362882 2543.03076315477 2478.78050186034 2415.26261793494 2352.4518486616 2290.32369278385 2228.85437473538 2168.02081061809 2107.80057582154 2048.17187418409 1989.11350860242;3687.49931828197 3604.02771170464 3521.73841154027 3440.59111634842 3360.54694541796 3281.56836896228 3203.61914215416 3126.66424274874 3050.66981206134 2975.60309908359 2901.43240753707 2828.12704567777 2755.6572786779 2683.9942834234 2613.11010557704 2542.97761876678 2473.57048576894 2404.8631215641 2336.83065815196 2269.44891101877;4143.00047553716 4049.21797528579 3956.76382674606 3865.59275021144 3775.66106220143 3686.92659703397 3599.34863271199 3512.88782084123 3427.50612031721 3343.16673453836 3259.83405191936 3177.4735894952 3096.05193942085 3015.5367181852 2935.89651837023 2857.10086279818 2779.12016091979 2701.92566730665 2625.48944211983 2549.78431343512;4598.50163279235 4494.40823886693 4391.78924195184 4290.59438407447 4190.77517898491 4092.28482510566 3995.07812326983 3899.11139893372 3804.34242857308 3710.73036999313 3618.23569630166 3526.82013331263 3436.44660016381 3347.079152947 3258.68293116342 3171.22410682959 3084.66983607064 2998.98821304921 2914.1482260877 2830.11971585147;5054.00279004754 4939.59850244808 4826.81465715762 4715.59601793749 4605.88929576838 4497.64305317735 4390.80761382767 4285.3349770262 4181.17873682896 4078.2940054479 3976.63734068395 3876.16667713006 3776.84126090677 3678.62158770879 3581.46934395661 3485.34735086099 ...(+2764 chars)]  tireParamSet=vdynPassCar.mat  plySteer=off  turnslip=off  PRESMAX=tireRL__SIMULATION__PRESMAX  PRESMIN=tireRL__SIMULATION__PRESMIN  FZMAX=tireRL__SIMULATION__FZMAX  FZMIN=tireRL__SIMULATION__FZMIN  VXLOW=tireRL__SIMULATION__VXLOW  KPUMAX=tireRL__SIMULATION__KPUMAX  KPUMIN=tireRL__SIMULATION__KPUMIN  ALPMAX=tireRL__SIMULATION__ALPMAX  ALPMIN=tireRL__SIMULATION__ALPMIN  CAMMAX=tireRL__SIMULATION__CAMMAX  CAMMIN=tireRL__SIMULATION__CAMMIN  LONGVL=tireRL__SIMULATION__LONGVL  omegao=INIT__initialvalues__omega0_Wheels_radps__3  br=tireRL__WHEEL__br_Nmsprad  UNLOADED_RADIUS=tireRL__WHEEL__TYRE_RADIUS_MOD  NOMPRES=tireRL__WHEEL__NORMPRES  FNOMIN=tireRL__WHEEL__FNOMIN  WIDTH=tireRL__DIMENSION__WIDTH  MASS=tireRL__INERTIAL__m_Wheel_kg  IYY=tireRL__INERTIAL__Iyy_Wheel_kgm2  GRAVITY=- VEH__Environment__a_Gravity_mps2  zo=INIT__initialvalues__z0_TireDeflection_m__3  zdoto=INIT__initialvalues__v0z_Wheels_mps__3  BREFF=tireRL__VERTICAL__BREFF  DREFF=tireRL__VERTICAL__DREFF  FREFF=tireRL__VERTICAL__FREFF  Q_RE0=tireRL__VERTICAL__Q_RE0  Q_V1=tireRL__VERTICAL__Q_V1  Q_V2=tireRL__VERTICAL__Q_V2  Q_FZ1=tireRL__VERTICAL__Q_FZ1  Q_FZ2=tireRL__VERTICAL__Q_FZ2  Q_FZ3=tireRL__VERTICAL__Q_FZ3  Q_FCX=tireRL__VERTICAL__Q_FCX  Q_FCY=tireRL__VERTICAL__Q_FCY  Q_FCY2=tireRL__VERTICAL__Q_FCY2  PFZ1=tireRL__VERTICAL__PFZ1  VERTICAL_STIFFNESS=tireRL__VERTICAL__VERTICAL_STIFFNESS  VERTICAL_DAMPING=tireRL__VERTICAL__VERTICAL_DAMPING  LONGITUDINAL_STIFFNESS=tireRL__STRUCTURAL__LONGITUDINAL_STIFFNESS  LATERAL_STIFFNESS=tireRL__STRUCTURAL__LATERAL_STIFFNESS  PCFX1=tireRL__STRUCTURAL__PCFX1  PCFX2=tireRL__STRUCTURAL__PCFX2  PCFX3=tireRL__STRUCTURAL__PCFX3  PCFY1=tireRL__STRUCTURAL__PCFY1  PCFY2=tireRL__STRUCTURAL__PCFY2  PCFY3=tireRL__STRUCTURAL__PCFY3  Q_RA1=tireRL__CONTACTPATCH__Q_RA1  Q_RA2=tireRL__CONTACTPATCH__Q_RA2  Q_RB1=tireRL__CONTACTPATCH__Q_RB1  Q_RB2=tireRL__CONTACTPATCH__Q_RB2  PCX1=tireRL__LONGITUDINAL__PCX1  PDX1=tireRL__LONGITUDINAL__PDX1  PDX2=tireRL__LONGITUDINAL__PDX2  PDX3=tireRL__LONGITUDINAL__PDX3  PEX1=tireRL__LONGITUDINAL__PEX1  PEX2=tireRL__LONGITUDINAL__PEX2  PEX3=tireRL__LONGITUDINAL__PEX3  PEX4=tireRL__LONGITUDINAL__PEX4  PKX1=tireRL__LONGITUDINAL__PKX1  PKX2=tireRL__LONGITUDINAL__PKX2  PKX3=tireRL__LONGITUDINAL__PKX3  PHX1=tireRL__LONGITUDINAL__PHX1  PHX2=tireRL__LONGITUDINAL__PHX2  PVX1=tireRL__LONGITUDINAL__PVX1  PVX2=tireRL__LONGITUDINAL__PVX2  PPX1=tireRL__LONGITUDINAL__PPX1  PPX2=tireRL__LONGITUDINAL__PPX2  PPX3=tireRL__LONGITUDINAL__PPX3  PPX4=tireRL__LONGITUDINAL__PPX4  RBX1=tireRL__LONGITUDINAL__RBX1  RBX2=tireRL__LONGITUDINAL__RBX2  RBX3=tireRL__LONGITUDINAL__RBX3  RCX1=tireRL__LONGITUDINAL__RCX1  REX1=tireRL__LONGITUDINAL__REX1  REX2=tireRL__LONGITUDINAL__REX2  RHX1=tireRL__LONGITUDINAL__RHX1  QSX1=tireRL__OVERTURNING__QSX1  QSX2=tireRL__OVERTURNING__QSX2  QSX3=tireRL__OVERTURNING__QSX3  QSX4=tireRL__OVERTURNING__QSX4  QSX5=tireRL__OVERTURNING__QSX5  QSX6=tireRL__OVERTURNING__QSX6  QSX7=tireRL__OVERTURNING__QSX7  QSX8=tireRL__OVERTURNING__QSX8  QSX9=tireRL__OVERTURNING__QSX9  QSX10=tireRL__OVERTURNING__QSX10  QSX11=tireRL__OVERTURNING__QSX11  QSX12=tireRL__OVERTURNING__QSX12  QSX13=tireRL__OVERTURNING__QSX13  QSX14=tireRL__OVERTURNING__QSX14  PPMX1=tireRL__OVERTURNING__PPMX1  PCY1=tireRL__LATERAL__PCY1  PDY1=tireRL__LATERAL__PDY1  PDY2=tireRL__LATERAL__PDY2  PDY3=tireRL__LATERAL__PDY3  PEY1=tireRL__LATERAL__PEY1  PEY2=tireRL__LATERAL__PEY2  PEY3=tireRL__LATERAL__PEY3  PEY4=tireRL__LATERAL__PEY4  PEY5=tireRL__LATERAL__PEY5  PKY1=tireRL__LATERAL__PKY1  PKY2=tireRL__LATERAL__PKY2  PKY3=tireRL__LATERAL__PKY3  PKY4=tireRL__LATERAL__PKY4  PKY5=tireRL__LATERAL__PKY5  PKY6=tireRL__LATERAL__PKY6  PKY7=tireRL__LATERAL__PKY7  PHY1=tireRL__LATERAL__PHY1  PHY2=tireRL__LATERAL__PHY2  PVY1=tireRL__LATERAL__PVY1  PVY2=tireRL__LATERAL__PVY2  PVY3=tireRL__LATERAL__PVY3  PVY4=tireRL__LATERAL__PVY4  PPY1=tireRL__LATERAL__PPY1  PPY2=tireRL__LATERAL__PPY2  PPY3=tireRL__LATERAL__PPY3  PPY4=tireRL__LATERAL__PPY4  PPY5=tireRL__LATERAL__PPY5  RBY1=tireRL__LATERAL__RBY1  RBY2=tireRL__LATERAL__RBY2  RBY3=tireRL__LATERAL__RBY3  RBY4=tireRL__LATERAL__RBY4  RCY1=tireRL__LATERAL__RCY1  REY1=tireRL__LATERAL__REY1  REY2=tireRL__LATERAL__REY2  RHY1=tireRL__LATERAL__RHY1  RHY2=tireRL__LATERAL__RHY2  RVY1=tireRL__LATERAL__RVY1  RVY2=tireRL__LATERAL__RVY2  RVY3=tireRL__LATERAL__RVY3  RVY4=tireRL__LATERAL__RVY4  RVY5=tireRL__LATERAL__RVY5  RVY6=tireRL__LATERAL__RVY6  QSY1=tireRL__ROLLING__QSY1  QSY2=tireRL__ROLLING__QSY2  QSY3=tireRL__ROLLING__QSY3  QSY4=tireRL__ROLLING__QSY4  QSY5=tireRL__ROLLING__QSY5  QSY6=tireRL__ROLLING__QSY6  QSY7=tireRL__ROLLING__QSY7  QSY8=tireRL__ROLLING__QSY8  QBZ1=tireRL__ALIGNING__QBZ1  QBZ2=tireRL__ALIGNING__QBZ2  QBZ3=tireRL__ALIGNING__QBZ3  QBZ4=tireRL__ALIGNING__QBZ4  QBZ5=tireRL__ALIGNING__QBZ5  QBZ6=tireRL__ALIGNING__QBZ6  QBZ9=tireRL__ALIGNING__QBZ9  QBZ10=tireRL__ALIGNING__QBZ10  QCZ1=tireRL__ALIGNING__QCZ1  QDZ1=tireRL__ALIGNING__QDZ1  QDZ2=tireRL__ALIGNING__QDZ2  QDZ3=tireRL__ALIGNING__QDZ3  QDZ4=tireRL__ALIGNING__QDZ4  QDZ6=tireRL__ALIGNING__QDZ6  QDZ7=tireRL__ALIGNING__QDZ7  QDZ8=tireRL__ALIGNING__QDZ8  QDZ9=tireRL__ALIGNING__QDZ9  QDZ10=tireRL__ALIGNING__QDZ10  QDZ11=tireRL__ALIGNING__QDZ11  QEZ1=tireRL__ALIGNING__QEZ1  QEZ2=tireRL__ALIGNING__QEZ2  QEZ3=tireRL__ALIGNING__QEZ3  QEZ4=tireRL__ALIGNING__QEZ4  QEZ5=tireRL__ALIGNING__QEZ5  QHZ1=tireRL__ALIGNING__QHZ1  QHZ2=tireRL__ALIGNING__QHZ2  QHZ3=tireRL__ALIGNING__QHZ3  QHZ4=tireRL__ALIGNING__QHZ4  PPZ1=tireRL__ALIGNING__PPZ1  PPZ2=tireRL__ALIGNING__PPZ2  SSZ1=tireRL__ALIGNING__SSZ1  SSZ2=tireRL__ALIGNING__SSZ2  SSZ3=tireRL__ALIGNING__SSZ3  SSZ4=tireRL__ALIGNING__SSZ4  PDXP1=tireRL__TURNSLIP__PDXP1  PDXP2=tireRL__TURNSLIP__PDXP2  PDXP3=tireRL__TURNSLIP__PDXP3  PKYP1=tireRL__TURNSLIP__PKYP1  PDYP1=tireRL__TURNSLIP__PDYP1  PDYP2=tireRL__TURNSLIP__PDYP2  PDYP3=tireRL__TURNSLIP__PDYP3  PDYP4=tireRL__TURNSLIP__PDYP4  PHYP1=tireRL__TURNSLIP__PHYP1  PHYP2=tireRL__TURNSLIP__PHYP2  PHYP3=tireRL__TURNSLIP__PHYP3  PHYP4=tireRL__TURNSLIP__PHYP4  PECP1=tireRL__TURNSLIP__PECP1  PECP2=tireRL__TURNSLIP__PECP2  QDTP1=tireRL__TURNSLIP__QDTP1  QCRP1=tireRL__TURNSLIP__QCRP1  QCRP2=tireRL__TURNSLIP__QCRP2  QBRP1=tireRL__TURNSLIP__QBRP1  QDRP1=tireRL__TURNSLIP__QDRP1  QDRP2=tireRL__TURNSLIP__QDRP2  aMode=2
  Combined Slip Wheel 2DOF - RearRight - TUM : vehdynlibtire_TUM/Combined Slip Wheel 2DOF  BrakeType=Disc  mu_static=VEH__Brakes__mue_BrakePadsFrRe_static__2  mu_kinetic=VEH__Brakes__mue_BrakePadsFrRe_kinetic__2  disk_abore=VEH__Brakes__d_BrakeActuatorBoreFrRe_m__2  Rm=VEH__Brakes__r_BrakePadsMeanLeverFrRe_m__2  num_pads=VEH__Brakes__n_BrakePadsNumberFrRe__2  drum_abore=0.0508  drum_a=0.123  drum_c=0.212  drum_r=0.15  drum_theta1=0  drum_theta2=126  brake_p_bpt=[1 11.4736842105263 21.9473684210526 32.4210526315789 42.8947368421053 53.3684210526316 63.8421052631579 74.3157894736842 84.7894736842105 95.2631578947368 105.736842105263 116.210526315789 126.684210526316 137.157894736842 147.631578947368 158.105263157895 168.578947368421 179.052631578947 189.526315789474 200]  brake_n_bpt=[0 52.6315789473684 105.263157894737 157.894736842105 210.526315789474 263.157894736842 315.789473684211 368.421052631579 421.052631578947 473.684210526316 526.315789473684 578.947368421053 631.578947368421 684.210526315789 736.842105263158 789.473684210526 842.105263157895 894.736842105263 947.368421052632 1000]  f_brake_t=[43.4900602404453 42.5056030554862 41.5350898940194 40.5780454442085 39.6340111501808 38.7025443887544 37.7832176914519 36.8756180088306 35.9793460143796 35.0940154454303 34.2192524787115 33.3546951383474 32.4999927342521 31.6548053290159 30.8188032315107 29.991666515561 29.1730845621415 28.362755623661 27.5603864089927 26.765691687993;498.991217495636 487.695866636631 476.560505099801 465.579679307235 454.748127933653 444.060772460445 433.51270824929 423.099196101319 412.81565427025 402.657650900201 392.620896861006 382.701238955775 372.894653477208 363.197240090814 353.605216024701 344.114910546964 334.722759712992 325.425301366216 316.219170376863 307.10109410434;954.492374750826 932.886130217776 911.585920305583 890.581313170261 869.862244717126 849.419000532136 829.242198807128 809.322774193808 789.651962526121 770.221286354971 751.0225412433 732.047782773203 713.289314220164 694.739674852612 676.391628817892 658.238154578366 640.272434863842 622.48784710877 604.877954344734 587.436496520688;1409.99353200602 1378.07639379892 1346.61133551136 1315.58294703329 1284.9763615006 1254.77722860383 1224.97168936497 1195.5463522863 1166.48827078199 1137.78492180974 1109.42418562559 1081.39432659063 1053.68397496312 1026.28210961441 999.178041611083 972.361398609768 945.822110014692 919.550392851325 893.536738312604 867.771898937035;1865.49468926121 1823.26665738007 1781.63675071715 1740.58458089631 1700.09047828407 1660.13545667552 1620.7011799228 1581.76993037878 1543.32457903786 1505.34855726451 1467.82583000789 1430.74087040806 1394.07863570608 1357.82454437621 1321.96445440427 1286.48464264117 1251.37178516554 1216.61293859388 1182.19552228048 1148.10730135338;2320.9958465164 2268.45692096121 2216.66216592293 2165.58621475934 2115.20459506754 2065.49368474721 2016.43067048064 1967.99350847127 1920.16088729373 1872.91219271928 1826.22747439018 1780.08741422549 1734.47329644903 1689.36697913801 1644.75086719747 1600.60788667257 1556.92146031639 1513.67548433643 1470.85430624835 1428.44270376973;2776.49700377159 2713.64718454235 2651.68758112871 2590.58784862237 2530.31871185102 2470.8519128189 2412.16016103848 2354.21708656376 2296.9971955496 2240.47582817405 2184.62911877248 2129.43395804292 2074.86795719199 2020.9094138998 1967.53727999066 1914.73113070398 1862.47113546724 1810.73803007899 1759.51309021622 1708.77810618608;3231.99816102678 3158.8374481235 3086.71299633449 3015.58948248539 2945.43282863449 2876.21014089059 2807.88965159632 2740.44066465625 2673.83350380547 2608.03946362882 2543.03076315477 2478.78050186034 2415.26261793494 2352.4518486616 2290.32369278385 2228.85437473538 2168.02081061809 2107.80057582154 2048.17187418409 1989.11350860242;3687.49931828197 3604.02771170464 3521.73841154027 3440.59111634842 3360.54694541796 3281.56836896228 3203.61914215416 3126.66424274874 3050.66981206134 2975.60309908359 2901.43240753707 2828.12704567777 2755.6572786779 2683.9942834234 2613.11010557704 2542.97761876678 2473.57048576894 2404.8631215641 2336.83065815196 2269.44891101877;4143.00047553716 4049.21797528579 3956.76382674606 3865.59275021144 3775.66106220143 3686.92659703397 3599.34863271199 3512.88782084123 3427.50612031721 3343.16673453836 3259.83405191936 3177.4735894952 3096.05193942085 3015.5367181852 2935.89651837023 2857.10086279818 2779.12016091979 2701.92566730665 2625.48944211983 2549.78431343512;4598.50163279235 4494.40823886693 4391.78924195184 4290.59438407447 4190.77517898491 4092.28482510566 3995.07812326983 3899.11139893372 3804.34242857308 3710.73036999313 3618.23569630166 3526.82013331263 3436.44660016381 3347.079152947 3258.68293116342 3171.22410682959 3084.66983607064 2998.98821304921 2914.1482260877 2830.11971585147;5054.00279004754 4939.59850244808 4826.81465715762 4715.59601793749 4605.88929576838 4497.64305317735 4390.80761382767 4285.3349770262 4181.17873682896 4078.2940054479 3976.63734068395 3876.16667713006 3776.84126090677 3678.62158770879 3581.46934395661 3485.34735086099 ...(+2764 chars)]  tireParamSet=vdynPassCar.mat  plySteer=off  turnslip=off  PRESMAX=tireRR__SIMULATION__PRESMAX  PRESMIN=tireRR__SIMULATION__PRESMIN  FZMAX=tireRR__SIMULATION__FZMAX  FZMIN=tireRR__SIMULATION__FZMIN  VXLOW=tireRR__SIMULATION__VXLOW  KPUMAX=tireRR__SIMULATION__KPUMAX  KPUMIN=tireRR__SIMULATION__KPUMIN  ALPMAX=tireRR__SIMULATION__ALPMAX  ALPMIN=tireRR__SIMULATION__ALPMIN  CAMMAX=tireRR__SIMULATION__CAMMAX  CAMMIN=tireRR__SIMULATION__CAMMIN  LONGVL=tireRR__SIMULATION__LONGVL  omegao=INIT__initialvalues__omega0_Wheels_radps__4  br=tireRR__WHEEL__br_Nmsprad  UNLOADED_RADIUS=tireRR__WHEEL__TYRE_RADIUS_MOD  NOMPRES=tireRR__WHEEL__NORMPRES  FNOMIN=tireRR__WHEEL__FNOMIN  WIDTH=tireRR__DIMENSION__WIDTH  MASS=tireRR__INERTIAL__m_Wheel_kg  IYY=tireRR__INERTIAL__Iyy_Wheel_kgm2  GRAVITY=- VEH__Environment__a_Gravity_mps2  zo=INIT__initialvalues__z0_TireDeflection_m__4  zdoto=INIT__initialvalues__v0z_Wheels_mps__4  BREFF=tireRR__VERTICAL__BREFF  DREFF=tireRR__VERTICAL__DREFF  FREFF=tireRR__VERTICAL__FREFF  Q_RE0=tireRR__VERTICAL__Q_RE0  Q_V1=tireRR__VERTICAL__Q_V1  Q_V2=tireRR__VERTICAL__Q_V2  Q_FZ1=tireRR__VERTICAL__Q_FZ1  Q_FZ2=tireRR__VERTICAL__Q_FZ2  Q_FZ3=tireRR__VERTICAL__Q_FZ3  Q_FCX=tireRR__VERTICAL__Q_FCX  Q_FCY=tireRR__VERTICAL__Q_FCY  Q_FCY2=tireRR__VERTICAL__Q_FCY2  PFZ1=tireRR__VERTICAL__PFZ1  VERTICAL_STIFFNESS=tireRR__VERTICAL__VERTICAL_STIFFNESS  VERTICAL_DAMPING=tireRR__VERTICAL__VERTICAL_DAMPING  LONGITUDINAL_STIFFNESS=tireRR__STRUCTURAL__LONGITUDINAL_STIFFNESS  LATERAL_STIFFNESS=tireRR__STRUCTURAL__LATERAL_STIFFNESS  PCFX1=tireRR__STRUCTURAL__PCFX1  PCFX2=tireRR__STRUCTURAL__PCFX2  PCFX3=tireRR__STRUCTURAL__PCFX3  PCFY1=tireRR__STRUCTURAL__PCFY1  PCFY2=tireRR__STRUCTURAL__PCFY2  PCFY3=tireRR__STRUCTURAL__PCFY3  Q_RA1=tireRR__CONTACTPATCH__Q_RA1  Q_RA2=tireRR__CONTACTPATCH__Q_RA2  Q_RB1=tireRR__CONTACTPATCH__Q_RB1  Q_RB2=tireRR__CONTACTPATCH__Q_RB2  PCX1=tireRR__LONGITUDINAL__PCX1  PDX1=tireRR__LONGITUDINAL__PDX1  PDX2=tireRR__LONGITUDINAL__PDX2  PDX3=tireRR__LONGITUDINAL__PDX3  PEX1=tireRR__LONGITUDINAL__PEX1  PEX2=tireRR__LONGITUDINAL__PEX2  PEX3=tireRR__LONGITUDINAL__PEX3  PEX4=tireRR__LONGITUDINAL__PEX4  PKX1=tireRR__LONGITUDINAL__PKX1  PKX2=tireRR__LONGITUDINAL__PKX2  PKX3=tireRR__LONGITUDINAL__PKX3  PHX1=tireRR__LONGITUDINAL__PHX1  PHX2=tireRR__LONGITUDINAL__PHX2  PVX1=tireRR__LONGITUDINAL__PVX1  PVX2=tireRR__LONGITUDINAL__PVX2  PPX1=tireRR__LONGITUDINAL__PPX1  PPX2=tireRR__LONGITUDINAL__PPX2  PPX3=tireRR__LONGITUDINAL__PPX3  PPX4=tireRR__LONGITUDINAL__PPX4  RBX1=tireRR__LONGITUDINAL__RBX1  RBX2=tireRR__LONGITUDINAL__RBX2  RBX3=tireRR__LONGITUDINAL__RBX3  RCX1=tireRR__LONGITUDINAL__RCX1  REX1=tireRR__LONGITUDINAL__REX1  REX2=tireRR__LONGITUDINAL__REX2  RHX1=tireRR__LONGITUDINAL__RHX1  QSX1=tireRR__OVERTURNING__QSX1  QSX2=tireRR__OVERTURNING__QSX2  QSX3=tireRR__OVERTURNING__QSX3  QSX4=tireRR__OVERTURNING__QSX4  QSX5=tireRR__OVERTURNING__QSX5  QSX6=tireRR__OVERTURNING__QSX6  QSX7=tireRR__OVERTURNING__QSX7  QSX8=tireRR__OVERTURNING__QSX8  QSX9=tireRR__OVERTURNING__QSX9  QSX10=tireRR__OVERTURNING__QSX10  QSX11=tireRR__OVERTURNING__QSX11  QSX12=tireRR__OVERTURNING__QSX12  QSX13=tireRR__OVERTURNING__QSX13  QSX14=tireRR__OVERTURNING__QSX14  PPMX1=tireRR__OVERTURNING__PPMX1  PCY1=tireRR__LATERAL__PCY1  PDY1=tireRR__LATERAL__PDY1  PDY2=tireRR__LATERAL__PDY2  PDY3=tireRR__LATERAL__PDY3  PEY1=tireRR__LATERAL__PEY1  PEY2=tireRR__LATERAL__PEY2  PEY3=tireRR__LATERAL__PEY3  PEY4=tireRR__LATERAL__PEY4  PEY5=tireRR__LATERAL__PEY5  PKY1=tireRR__LATERAL__PKY1  PKY2=tireRR__LATERAL__PKY2  PKY3=tireRR__LATERAL__PKY3  PKY4=tireRR__LATERAL__PKY4  PKY5=tireRR__LATERAL__PKY5  PKY6=tireRR__LATERAL__PKY6  PKY7=tireRR__LATERAL__PKY7  PHY1=tireRR__LATERAL__PHY1  PHY2=tireRR__LATERAL__PHY2  PVY1=tireRR__LATERAL__PVY1  PVY2=tireRR__LATERAL__PVY2  PVY3=tireRR__LATERAL__PVY3  PVY4=tireRR__LATERAL__PVY4  PPY1=tireRR__LATERAL__PPY1  PPY2=tireRR__LATERAL__PPY2  PPY3=tireRR__LATERAL__PPY3  PPY4=tireRR__LATERAL__PPY4  PPY5=tireRR__LATERAL__PPY5  RBY1=tireRR__LATERAL__RBY1  RBY2=tireRR__LATERAL__RBY2  RBY3=tireRR__LATERAL__RBY3  RBY4=tireRR__LATERAL__RBY4  RCY1=tireRR__LATERAL__RCY1  REY1=tireRR__LATERAL__REY1  REY2=tireRR__LATERAL__REY2  RHY1=tireRR__LATERAL__RHY1  RHY2=tireRR__LATERAL__RHY2  RVY1=tireRR__LATERAL__RVY1  RVY2=tireRR__LATERAL__RVY2  RVY3=tireRR__LATERAL__RVY3  RVY4=tireRR__LATERAL__RVY4  RVY5=tireRR__LATERAL__RVY5  RVY6=tireRR__LATERAL__RVY6  QSY1=tireRR__ROLLING__QSY1  QSY2=tireRR__ROLLING__QSY2  QSY3=tireRR__ROLLING__QSY3  QSY4=tireRR__ROLLING__QSY4  QSY5=tireRR__ROLLING__QSY5  QSY6=tireRR__ROLLING__QSY6  QSY7=tireRR__ROLLING__QSY7  QSY8=tireRR__ROLLING__QSY8  QBZ1=tireRR__ALIGNING__QBZ1  QBZ2=tireRR__ALIGNING__QBZ2  QBZ3=tireRR__ALIGNING__QBZ3  QBZ4=tireRR__ALIGNING__QBZ4  QBZ5=tireRR__ALIGNING__QBZ5  QBZ6=tireRR__ALIGNING__QBZ6  QBZ9=tireRR__ALIGNING__QBZ9  QBZ10=tireRR__ALIGNING__QBZ10  QCZ1=tireRR__ALIGNING__QCZ1  QDZ1=tireRR__ALIGNING__QDZ1  QDZ2=tireRR__ALIGNING__QDZ2  QDZ3=tireRR__ALIGNING__QDZ3  QDZ4=tireRR__ALIGNING__QDZ4  QDZ6=tireRR__ALIGNING__QDZ6  QDZ7=tireRR__ALIGNING__QDZ7  QDZ8=tireRR__ALIGNING__QDZ8  QDZ9=tireRR__ALIGNING__QDZ9  QDZ10=tireRR__ALIGNING__QDZ10  QDZ11=tireRR__ALIGNING__QDZ11  QEZ1=tireRR__ALIGNING__QEZ1  QEZ2=tireRR__ALIGNING__QEZ2  QEZ3=tireRR__ALIGNING__QEZ3  QEZ4=tireRR__ALIGNING__QEZ4  QEZ5=tireRR__ALIGNING__QEZ5  QHZ1=tireRR__ALIGNING__QHZ1  QHZ2=tireRR__ALIGNING__QHZ2  QHZ3=tireRR__ALIGNING__QHZ3  QHZ4=tireRR__ALIGNING__QHZ4  PPZ1=tireRR__ALIGNING__PPZ1  PPZ2=tireRR__ALIGNING__PPZ2  SSZ1=tireRR__ALIGNING__SSZ1  SSZ2=tireRR__ALIGNING__SSZ2  SSZ3=tireRR__ALIGNING__SSZ3  SSZ4=tireRR__ALIGNING__SSZ4  PDXP1=tireRR__TURNSLIP__PDXP1  PDXP2=tireRR__TURNSLIP__PDXP2  PDXP3=tireRR__TURNSLIP__PDXP3  PKYP1=tireRR__TURNSLIP__PKYP1  PDYP1=tireRR__TURNSLIP__PDYP1  PDYP2=tireRR__TURNSLIP__PDYP2  PDYP3=tireRR__TURNSLIP__PDYP3  PDYP4=tireRR__TURNSLIP__PDYP4  PHYP1=tireRR__TURNSLIP__PHYP1  PHYP2=tireRR__TURNSLIP__PHYP2  PHYP3=tireRR__TURNSLIP__PHYP3  PHYP4=tireRR__TURNSLIP__PHYP4  PECP1=tireRR__TURNSLIP__PECP1  PECP2=tireRR__TURNSLIP__PECP2  QDTP1=tireRR__TURNSLIP__QDTP1  QCRP1=tireRR__TURNSLIP__QCRP1  QCRP2=tireRR__TURNSLIP__QCRP2  QBRP1=tireRR__TURNSLIP__QBRP1  QDRP1=tireRR__TURNSLIP__QDRP1  QDRP2=tireRR__TURNSLIP__QDRP2  aMode=2
  Fx : Subsystem
  Fy : Subsystem
  Fz : Subsystem
  Mx : Subsystem
  My : Subsystem
  Mz : Subsystem
  Re : Subsystem
  Selector{,1..8} (9 alike) : Selector  InputPortWidth=4  IndexOptions=Index vector (dialog)  Indices=1  OutputSizes=1
  Selector{10..18} (9 alike) : Selector  InputPortWidth=4  IndexOptions=Index vector (dialog)  Indices=2  OutputSizes=1
  Selector19 : Selector  NumberOfDimensions=2  InputPortWidth=4  IndexOptions=Select all,Index vector (dialog)  Indices=1,2  OutputSizes=1,1
  Selector{20..28} (9 alike) : Selector  InputPortWidth=4  IndexOptions=Index vector (dialog)  Indices=3  OutputSizes=1
  Selector29 : Selector  NumberOfDimensions=2  InputPortWidth=4  IndexOptions=Select all,Index vector (dialog)  Indices=1,3  OutputSizes=1,1
  Selector{30..38} (9 alike) : Selector  InputPortWidth=4  IndexOptions=Index vector (dialog)  Indices=4  OutputSizes=1
  Selector39 : Selector  NumberOfDimensions=2  InputPortWidth=4  IndexOptions=Select all,Index vector (dialog)  Indices=1,4  OutputSizes=1,1
  Selector9 : Selector  NumberOfDimensions=2  InputPortWidth=4  IndexOptions=Select all,Index vector (dialog)  Indices=1,1  OutputSizes=1,1
  Signal Specification{,1..3} (4 alike) : SignalSpecification  Unit=1
  Terminator{,1..27} (28 alike) : Terminator
  alpha : Subsystem
  kappa : Subsystem
  omega : Subsystem
  z : Subsystem
  zdot : Subsystem
  Wheels : Outport
  wires:
  Bus Creator/1 -> Wheels/1
  Brake Pressure/1 -> Selector30/1, Selector20/1, Selector10/1, Selector/1
  DriveTorque/1 -> Selector31/1, Selector21/1, Selector11/1, Selector1/1
  Vx/1 -> Selector12/1, Selector32/1, Selector22/1, Selector2/1
  Selector/1 -> Combined Slip Wheel 2DOF - FrontLeft - TUM/1
  Selector1/1 -> Combined Slip Wheel 2DOF - FrontLeft - TUM/2
  Selector7/1 -> Combined Slip Wheel 2DOF - FrontLeft - TUM/8
  Selector6/1 -> Combined Slip Wheel 2DOF - FrontLeft - TUM/7
  Selector5/1 -> Combined Slip Wheel 2DOF - FrontLeft - TUM/6
  Selector4/1 -> Combined Slip Wheel 2DOF - FrontLeft - TUM/5
  Selector9/1 -> Signal Specification/1
  Selector8/1 -> Combined Slip Wheel 2DOF - FrontLeft - TUM/9
  Camber/1 -> Selector34/1, Selector24/1, Selector14/1, Selector4/1
  Vy/1 -> Selector33/1, Selector23/1, Selector13/1, Selector3/1
  r/1 -> Selector15/1, Selector35/1, Selector25/1, Selector5/1
  Press/1 -> Selector36/1, Selector26/1, Selector16/1, Selector6/1
  Gnd/1 -> Selector37/1, Selector27/1, Selector17/1, Selector7/1
  FzSusp/1 -> Selector38/1, Selector28/1, Selector18/1, Selector8/1
  lambda/1 -> Selector9/1, Selector19/1, Selector39/1, Selector29/1
  Selector18/1 -> Combined Slip Wheel 2DOF - FrontRight - TUM/9
  Selector19/1 -> Signal Specification1/1
  Selector14/1 -> Combined Slip Wheel 2DOF - FrontRight - TUM/5
  Selector15/1 -> Combined Slip Wheel 2DOF - FrontRight - TUM/6
  Selector16/1 -> Combined Slip Wheel 2DOF - FrontRight - TUM/7
  Selector17/1 -> Combined Slip Wheel 2DOF - FrontRight - TUM/8
  Selector12/1 -> Combined Slip Wheel 2DOF - FrontRight - TUM/3
  Selector13/1 -> Combined Slip Wheel 2DOF - FrontRight - TUM/4
  Selector11/1 -> Combined Slip Wheel 2DOF - FrontRight - TUM/2
  Selector10/1 -> Combined Slip Wheel 2DOF - FrontRight - TUM/1
  Selector30/1 -> Combined Slip Wheel 2DOF - RearRight - TUM/1
  Selector31/1 -> Combined Slip Wheel 2DOF - RearRight - TUM/2
  Selector33/1 -> Combined Slip Wheel 2DOF - RearRight - TUM/4
  Selector32/1 -> Combined Slip Wheel 2DOF - RearRight - TUM/3
  Selector37/1 -> Combined Slip Wheel 2DOF - RearRight - TUM/8
  Selector36/1 -> Combined Slip Wheel 2DOF - RearRight - TUM/7
  Selector35/1 -> Combined Slip Wheel 2DOF - RearRight - TUM/6
  Selector34/1 -> Combined Slip Wheel 2DOF - RearRight - TUM/5
  Selector39/1 -> Signal Specification3/1
  Selector38/1 -> Combined Slip Wheel 2DOF - RearRight - TUM/9
  Selector28/1 -> Combined Slip Wheel 2DOF - RearLeft - TUM/9
  Selector29/1 -> Signal Specification2/1
  Selector24/1 -> Combined Slip Wheel 2DOF - RearLeft - TUM/5
  Selector25/1 -> Combined Slip Wheel 2DOF - RearLeft - TUM/6
  Selector26/1 -> Combined Slip Wheel 2DOF - RearLeft - TUM/7
  Selector27/1 -> Combined Slip Wheel 2DOF - RearLeft - TUM/8
  Selector22/1 -> Combined Slip Wheel 2DOF - RearLeft - TUM/3
  Selector23/1 -> Combined Slip Wheel 2DOF - RearLeft - TUM/4
  Selector21/1 -> Combined Slip Wheel 2DOF - RearLeft - TUM/2
  Selector20/1 -> Combined Slip Wheel 2DOF - RearLeft - TUM/1
  Combined Slip Wheel 2DOF - FrontRight - TUM/1 -> omega/2(In2), Fx/2(In2), Mx/2(In2), My/2(In2), alpha/2(In2), kappa/2(In2), zdot/2(In2), z/2(In2), Re/2(In2), Mz/2(In2), Fz/2(In2), Fy/2(In2)
  Combined Slip Wheel 2DOF - RearLeft - TUM/1 -> My/3(In3), alpha/3(In3), kappa/3(In3), zdot/3(In3), z/3(In3), Re/3(In3), Mz/3(In3), Mx/3(In3), Fz/3(In3), Fy/3(In3), Fx/3(In3), omega/3(In3)
  Combined Slip Wheel 2DOF - RearRight - TUM/1 -> omega/4(In4), Fx/4(In4), Fy/4(In4), Fz/4(In4), Mx/4(In4), My/4(In4), Mz/4(In4), Re/4(In4), z/4(In4), zdot/4(In4), kappa/4(In4), alpha/4(In4)
  Combined Slip Wheel 2DOF - FrontLeft - TUM/1 -> Mx/1(In1), My/1(In1), alpha/1(In1), kappa/1(In1), zdot/1(In1), z/1(In1), Re/1(In1), Mz/1(In1), Fz/1(In1), Fy/1(In1), Fx/1(In1), omega/1(In1)
  omega/1(Out1) -> Bus Creator/1  "omega"
  Fx/1(Out1) -> Bus Creator/2  "Fx"
  Mz/1(Out1) -> Bus Creator/7  "Mz"
  Fz/1(Out1) -> Bus Creator/4  "Fz"
  Re/1(Out1) -> Bus Creator/8  "Re"
  z/1(Out1) -> Bus Creator/9  "z"
  zdot/1(Out1) -> Bus Creator/10  "zdot"
  Mx/1(Out1) -> Bus Creator/5  "Mx"
  My/1(Out1) -> Bus Creator/6  "My"
  kappa/1(Out1) -> Bus Creator/11  "Kappa"
  Fy/1(Out1) -> Bus Creator/3  "Fy"
  Selector2/1 -> Combined Slip Wheel 2DOF - FrontLeft - TUM/3
  Selector3/1 -> Combined Slip Wheel 2DOF - FrontLeft - TUM/4
  Signal Specification/1 -> Combined Slip Wheel 2DOF - FrontLeft - TUM/10
  Signal Specification1/1 -> Combined Slip Wheel 2DOF - FrontRight - TUM/10
  Signal Specification2/1 -> Combined Slip Wheel 2DOF - RearLeft - TUM/10
  Signal Specification3/1 -> Combined Slip Wheel 2DOF - RearRight - TUM/10
  Combined Slip Wheel 2DOF - FrontLeft - TUM/2 -> Terminator/1
  Combined Slip Wheel 2DOF - FrontLeft - TUM/3 -> Terminator1/1
  Combined Slip Wheel 2DOF - FrontLeft - TUM/4 -> Terminator2/1
  Combined Slip Wheel 2DOF - FrontLeft - TUM/7 -> Terminator5/1
  Combined Slip Wheel 2DOF - FrontLeft - TUM/6 -> Terminator4/1
  Combined Slip Wheel 2DOF - FrontLeft - TUM/5 -> Terminator3/1
  Combined Slip Wheel 2DOF - FrontLeft - TUM/8 -> Terminator6/1
  Combined Slip Wheel 2DOF - FrontRight - TUM/2 -> Terminator7/1
  Combined Slip Wheel 2DOF - FrontRight - TUM/3 -> Terminator8/1
  Combined Slip Wheel 2DOF - FrontRight - TUM/4 -> Terminator9/1
  Combined Slip Wheel 2DOF - FrontRight - TUM/5 -> Terminator10/1
  Combined Slip Wheel 2DOF - FrontRight - TUM/6 -> Terminator11/1
  Combined Slip Wheel 2DOF - FrontRight - TUM/7 -> Terminator12/1
  Combined Slip Wheel 2DOF - FrontRight - TUM/8 -> Terminator13/1
  Combined Slip Wheel 2DOF - RearLeft - TUM/2 -> Terminator18/1
  Combined Slip Wheel 2DOF - RearLeft - TUM/3 -> Terminator19/1
  Combined Slip Wheel 2DOF - RearLeft - TUM/4 -> Terminator20/1
  Combined Slip Wheel 2DOF - RearLeft - TUM/5 -> Terminator14/1
  Combined Slip Wheel 2DOF - RearLeft - TUM/6 -> Terminator15/1
  Combined Slip Wheel 2DOF - RearLeft - TUM/7 -> Terminator16/1
  Combined Slip Wheel 2DOF - RearLeft - TUM/8 -> Terminator17/1
  Combined Slip Wheel 2DOF - RearRight - TUM/2 -> Terminator25/1
  Combined Slip Wheel 2DOF - RearRight - TUM/3 -> Terminator26/1
  Combined Slip Wheel 2DOF - RearRight - TUM/4 -> Terminator27/1
  Combined Slip Wheel 2DOF - RearRight - TUM/5 -> Terminator21/1
  Combined Slip Wheel 2DOF - RearRight - TUM/6 -> Terminator22/1
  Combined Slip Wheel 2DOF - RearRight - TUM/7 -> Terminator23/1
  Combined Slip Wheel 2DOF - RearRight - TUM/8 -> Terminator24/1
  alpha/1(Out1) -> Bus Creator/12  "Alpha"
